simulink model "arte"  (R2013b)
settings: Solver=ode45  StartTime=0.0  StopTime=10.0  RelTol=1e-3
undefined symbols (not defined in the file or in its folder): sfp
libraries: xbsIndex_r4 x3084, casper_library_delays x44, casper_library_misc x20, dspsigops x16, xps_library x7, simulink x3
(part 1 of 27)
settings Model: Creator=root  LastModifiedBy=root
settings DebuggingCC: StateNameClashWarn=warning

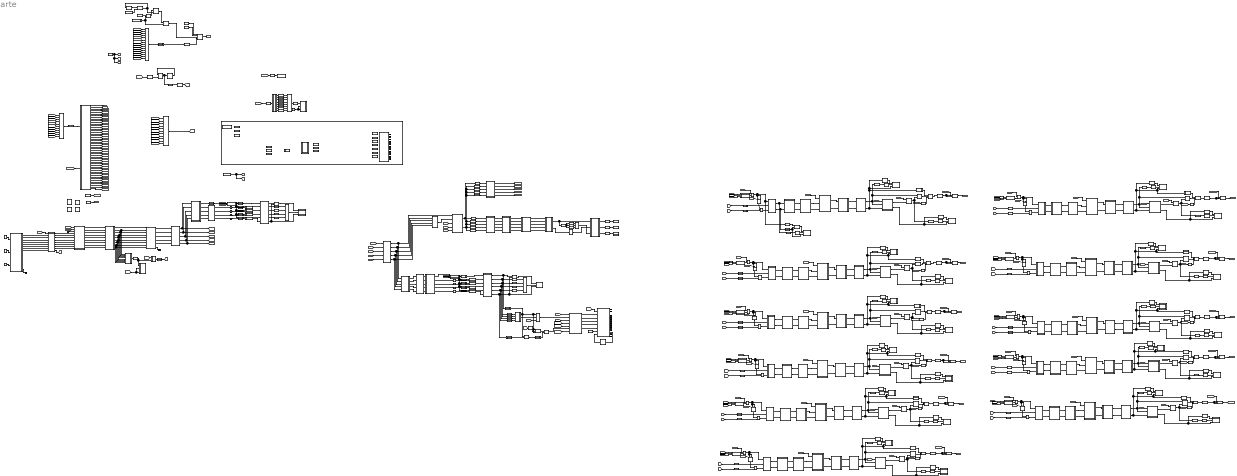
== system arte ==
  note: 5000--> 1
  note: add:3, mul:5 ->17k
  note: add:5, mul:3 ->856
  note: check if we could
      | hardcode the gain
  note: meanwhile
      | header
  note: 0xaabbccdd
  note: DRAM ring buffer + 1gbeth dump
  note: le puse un rst al contador del read!!! revisar
  " System Generator" : xbsIndex_r4/ System Generator  Tag=genX  xilinxfamily=virtex6  part=xc6vsx475t  speed=-1  package=ff1759  synthesis_tool=XST  clock_wrapper=Clock Enables  directory=./arte/sysgen  proj_type=Project Navigator  Synth_file=XST Defaults  Impl_file=ISE Defaults  testbench=off  simulink_period=1  sysclk_period=6.6667  dcm_input_clock_period=100  incr_netlist=off  trim_vbits=Everywhere in SubSystem  dbl_ovrd=According to Block Masks  core_generation=According to Block Masks  run_coregen=off  deprecated_control=off  eval_field=0  block_type=sysgen
  AddSub : xbsIndex_r4/AddSub  mode=Addition  use_carryin=off  use_carryout=off  en=off  latency=0  precision=User Defined  arith_type=Unsigned  n_bits=32  bin_pt=0  quantization=Truncate  overflow=Wrap  dbl_ovrd=off  use_behavioral_HDL=off  hw_selection=Fabric  pipelined=off  block_type=addsub
  Band-Limited White Noise : simulink/Sources/Band-Limited White Noise  Cov=[0.1]  Ts=0.1  seed=[23341]
  Band-Limited White Noise2 : simulink/Sources/Band-Limited White Noise  Cov=[0.1]  Ts=0.1  seed=[23341]
  Black Box5 : xbsIndex_r4/Black Box  init_code=fft_channel_flag_top_config  sim_method=Inactive  verbose=off  block_type=blackbox2
  Black Box6 : xbsIndex_r4/Black Box  init_code=pfb_fft_8in_2048ch_config  sim_method=Inactive  verbose=off  block_type=blackbox2
  Concat : xbsIndex_r4/Concat  num_inputs=4  dbl_ovrd=off  block_type=concat
  Concat10 : xbsIndex_r4/Concat  num_inputs=15  dbl_ovrd=off  block_type=concat
  Concat4 : xbsIndex_r4/Concat  num_inputs=4  dbl_ovrd=off  block_type=concat
  Concat5 : xbsIndex_r4/Concat  num_inputs=4  dbl_ovrd=off  block_type=concat
  Concat6 : xbsIndex_r4/Concat  num_inputs=3  dbl_ovrd=off  block_type=concat
  Concat9 : xbsIndex_r4/Concat  num_inputs=11  dbl_ovrd=off  block_type=concat
  Constant : xbsIndex_r4/Constant  const=2864434397  gui_display_data_type=Fixed-point  arith_type=Unsigned  n_bits=32  bin_pt=0  preci_type=Single  exp_width=8  frac_width=24  explicit_period=on  period=1  equ=P=C  opselect=C  inp2=PCIN>>17  opr=+  inp1=P  carry=CIN  dbl_ovrd=off  block_type=constant
  Constant1 : xbsIndex_r4/Constant  const=2864434397  gui_display_data_type=Fixed-point  arith_type=Unsigned  n_bits=32  bin_pt=0  preci_type=Single  exp_width=8  frac_width=24  explicit_period=on  period=1  equ=P=C  opselect=C  inp2=PCIN>>17  opr=+  inp1=P  carry=CIN  dbl_ovrd=off  block_type=constant
  Constant105 : xbsIndex_r4/Constant  const=1  gui_display_data_type=Boolean  arith_type=Boolean  n_bits=16  bin_pt=14  preci_type=Single  exp_width=8  frac_width=24  explicit_period=on  period=1  equ=P=C  opselect=C  inp2=PCIN>>17  opr=+  inp1=P  carry=CIN  dbl_ovrd=off  block_type=constant
  Constant13 : Constant
  Constant2 : xbsIndex_r4/Constant  const=2864434397  gui_display_data_type=Fixed-point  arith_type=Unsigned  n_bits=32  bin_pt=0  preci_type=Single  exp_width=8  frac_width=24  explicit_period=on  period=1  equ=P=C  opselect=C  inp2=PCIN>>17  opr=+  inp1=P  carry=CIN  dbl_ovrd=off  block_type=constant
  Constant3 : xbsIndex_r4/Constant  const=0  gui_display_data_type=Boolean  arith_type=Boolean  n_bits=16  bin_pt=14  preci_type=Single  exp_width=8  frac_width=24  explicit_period=on  period=1  equ=P=C  opselect=C  inp2=PCIN>>17  opr=+  inp1=P  carry=CIN  dbl_ovrd=off  block_type=constant
  Constant4 : xbsIndex_r4/Constant  const=1  gui_display_data_type=Boolean  arith_type=Boolean  n_bits=12  bin_pt=0  preci_type=Single  exp_width=8  frac_width=24  explicit_period=on  period=1  equ=P=C  opselect=C  inp2=PCIN>>17  opr=+  inp1=P  carry=CIN  dbl_ovrd=off  block_type=constant
  Constant5 : xbsIndex_r4/Constant  const=150*10^6  gui_display_data_type=Fixed-point  arith_type=Unsigned  n_bits=32  bin_pt=0  preci_type=Single  exp_width=8  frac_width=24  explicit_period=on  period=1  equ=P=C  opselect=C  inp2=PCIN>>17  opr=+  inp1=P  carry=CIN  dbl_ovrd=off  block_type=constant
  Constant6 : xbsIndex_r4/Constant  const=1  gui_display_data_type=Boolean  arith_type=Boolean  n_bits=16  bin_pt=14  preci_type=Single  exp_width=8  frac_width=24  explicit_period=on  period=1  equ=P=C  opselect=C  inp2=PCIN>>17  opr=+  inp1=P  carry=CIN  dbl_ovrd=off  block_type=constant
  Constant7 : xbsIndex_r4/Constant  const=0  gui_display_data_type=Fixed-point  arith_type=Unsigned  n_bits=32  bin_pt=0  preci_type=Single  exp_width=8  frac_width=24  explicit_period=on  period=1  equ=P=C  opselect=C  inp2=PCIN>>17  opr=+  inp1=P  carry=CIN  dbl_ovrd=off  block_type=constant
  Constant8 : xbsIndex_r4/Constant  const=1  gui_display_data_type=Boolean  arith_type=Boolean  n_bits=16  bin_pt=14  preci_type=Single  exp_width=8  frac_width=24  explicit_period=on  period=1  equ=P=C  opselect=C  inp2=PCIN>>17  opr=+  inp1=P  carry=CIN  dbl_ovrd=off  block_type=constant
  Constant9 : xbsIndex_r4/Constant  const=0  gui_display_data_type=Boolean  arith_type=Boolean  n_bits=16  bin_pt=14  preci_type=Single  exp_width=8  frac_width=24  explicit_period=on  period=1  equ=P=C  opselect=C  inp2=PCIN>>17  opr=+  inp1=P  carry=CIN  dbl_ovrd=off  block_type=constant
  Convert{1,3..4,6..13,22,31..40} (22 alike) : xbsIndex_r4/Convert  gui_display_data_type=Fixed-point  arith_type=Unsigned  n_bits=32  bin_pt=15  float_type=Single  exp_bits=8  fraction_bits=24  quantization=Truncate  overflow=Wrap  en=off  latency=0  dbl_ovrd=off  pipeline=off  block_type=convert
      settings: block_version=11.4
  Convert2 : xbsIndex_r4/Convert  gui_display_data_type=Fixed-point  arith_type="Signed  (2's comp)"  n_bits=32  bin_pt=15  float_type=Single  exp_bits=8  fraction_bits=24  quantization=Truncate  overflow=Wrap  en=off  latency=2  dbl_ovrd=off  pipeline=off  block_type=convert
      settings: block_version=11.4
  Convert{23..30} (8 alike) : xbsIndex_r4/Convert  gui_display_data_type=Fixed-point  arith_type="Signed  (2's comp)"  n_bits=8  bin_pt=0  float_type=Single  exp_bits=8  fraction_bits=24  quantization=Truncate  overflow=Wrap  en=off  latency=2  dbl_ovrd=off  pipeline=off  block_type=convert
      settings: block_version=11.4
  Convert41 : xbsIndex_r4/Convert  gui_display_data_type=Fixed-point  arith_type=Unsigned  n_bits=32  bin_pt=0  float_type=Single  exp_bits=8  fraction_bits=24  quantization=Truncate  overflow=Wrap  en=off  latency=2  dbl_ovrd=off  pipeline=off  block_type=convert
      settings: block_version=11.4
  Convert46 : xbsIndex_r4/Convert  gui_display_data_type=Boolean  arith_type=Boolean  n_bits=3  bin_pt=0  float_type=Single  exp_bits=8  fraction_bits=24  quantization=Truncate  overflow=Wrap  en=off  latency=0  dbl_ovrd=off  pipeline=off  block_type=convert
      settings: block_version=11.4
  Convert5 : xbsIndex_r4/Convert  gui_display_data_type=Boolean  arith_type=Boolean  n_bits=3  bin_pt=0  float_type=Single  exp_bits=8  fraction_bits=24  quantization=Truncate  overflow=Wrap  en=off  latency=0  dbl_ovrd=off  pipeline=off  block_type=convert
      settings: block_version=11.4
  Counter : xbsIndex_r4/Counter  cnt_type=Free Running  cnt_to=Inf  operation=Up  start_count=0  cnt_by_val=1  arith_type=Unsigned  n_bits=32  bin_pt=0  load_pin=off  rst=on  en=off  explicit_period=on  period=1  dbl_ovrd=off  use_behavioral_HDL=off  implementation=Fabric  block_type=counter
  Counter1 : xbsIndex_r4/Counter  cnt_type=Free Running  cnt_to=Inf  operation=Up  start_count=0  cnt_by_val=1  arith_type=Unsigned  n_bits=9  bin_pt=0  load_pin=off  rst=on  en=on  explicit_period=on  period=1  dbl_ovrd=off  use_behavioral_HDL=off  implementation=Fabric  block_type=counter
  Counter{8..9,12..19,21..32} (22 alike) : xbsIndex_r4/Counter  cnt_type=Free Running  cnt_to=Inf  operation=Up  start_count=0  cnt_by_val=1  arith_type=Unsigned  n_bits=10  bin_pt=0  load_pin=off  rst=off  en=on  explicit_period=on  period=1  dbl_ovrd=off  use_behavioral_HDL=off  implementation=Fabric  block_type=counter
  Counter33 : xbsIndex_r4/Counter  cnt_type=Free Running  cnt_to=Inf  operation=Up  start_count=0  cnt_by_val=1  arith_type=Unsigned  n_bits=28  bin_pt=0  load_pin=off  rst=on  en=off  explicit_period=on  period=1  dbl_ovrd=off  use_behavioral_HDL=off  implementation=Fabric  block_type=counter
  Counter34 : xbsIndex_r4/Counter  cnt_type=Free Running  cnt_to=Inf  operation=Up  start_count=0  cnt_by_val=1  arith_type=Unsigned  n_bits=32  bin_pt=0  load_pin=off  rst=on  en=on  explicit_period=on  period=1  dbl_ovrd=off  use_behavioral_HDL=off  implementation=Fabric  block_type=counter
  Counter5 : xbsIndex_r4/Counter  cnt_type=Free Running  cnt_to=Inf  operation=Up  start_count=0  cnt_by_val=1  arith_type=Unsigned  n_bits=9  bin_pt=0  load_pin=off  rst=on  en=on  explicit_period=on  period=1  dbl_ovrd=off  use_behavioral_HDL=off  implementation=Fabric  block_type=counter
  Counter6 : xbsIndex_r4/Counter  cnt_type=Free Running  cnt_to=Inf  operation=Up  start_count=0  cnt_by_val=1  arith_type=Unsigned  n_bits=3  bin_pt=0  load_pin=off  rst=on  en=off  explicit_period=on  period=1  dbl_ovrd=off  use_behavioral_HDL=off  implementation=Fabric  block_type=counter
  Counter7 : xbsIndex_r4/Counter  cnt_type=Free Running  cnt_to=Inf  operation=Up  start_count=0  cnt_by_val=1  arith_type=Unsigned  n_bits=6  bin_pt=0  load_pin=off  rst=on  en=on  explicit_period=on  period=1  dbl_ovrd=off  use_behavioral_HDL=off  implementation=Fabric  block_type=counter
  Delay{,2..5,32,34..36} (9 alike) : xbsIndex_r4/Delay  rst=off  infoeditControl=Selection of Reset will increase slice count due to use of real FFs and instead of SRLs  en=off  latency=1  dbl_ovrd=off  reg_retiming=off  block_type=delay
  Delay11 : xbsIndex_r4/Delay  rst=off  infoeditControl=Selection of Reset will increase slice count due to use of real FFs and instead of SRLs  en=off  latency=2  dbl_ovrd=off  reg_retiming=off  block_type=delay
  Delay49 : xbsIndex_r4/Delay  rst=off  infoeditControl=Selection of Reset will increase slice count due to use of real FFs and instead of SRLs  en=off  latency=2  dbl_ovrd=off  reg_retiming=off  block_type=delay
  Delay6 : xbsIndex_r4/Delay  rst=off  infoeditControl=Selection of Reset will increase slice count due to use of real FFs and instead of SRLs  en=off  latency=2  dbl_ovrd=off  reg_retiming=off  block_type=delay
  Delay91 : xbsIndex_r4/Delay  rst=off  infoeditControl=Selection of Reset will increase slice count due to use of real FFs and instead of SRLs  en=off  latency=3  dbl_ovrd=off  reg_retiming=off  block_type=delay
  Delay92 : xbsIndex_r4/Delay  rst=off  infoeditControl=Selection of Reset will increase slice count due to use of real FFs and instead of SRLs  en=off  latency=3  dbl_ovrd=off  reg_retiming=off  block_type=delay
  Delay93 : xbsIndex_r4/Delay  rst=off  infoeditControl=Selection of Reset will increase slice count due to use of real FFs and instead of SRLs  en=off  latency=3  dbl_ovrd=off  reg_retiming=off  block_type=delay
  Inverter : xbsIndex_r4/Inverter  en=off  latency=0  dbl_ovrd=off  block_type=inv
  Inverter{2,4..13} (11 alike) : xbsIndex_r4/Inverter  en=off  latency=1  dbl_ovrd=off  block_type=inv
  Inverter3 : xbsIndex_r4/Inverter  en=off  latency=0  dbl_ovrd=off  block_type=inv
  Logical : xbsIndex_r4/Logical  logical_function=OR  inputs=2  en=off  latency=0  precision=Full  arith_type=Unsigned  n_bits=16  bin_pt=0  align_bp=on  dbl_ovrd=off  block_type=logical
  Logical{1,16..22,24..27,29..30,32..33,35..36,38..39,41..42,44..45} (24 alike) : xbsIndex_r4/Logical  logical_function=AND  inputs=2  en=off  latency=0  precision=Full  arith_type=Unsigned  n_bits=16  bin_pt=0  align_bp=on  dbl_ovrd=off  block_type=logical
  Logical{2,11..15,28,31,34,37,40,43} (12 alike) : xbsIndex_r4/Logical  logical_function=AND  inputs=3  en=off  latency=0  precision=Full  arith_type=Unsigned  n_bits=16  bin_pt=0  align_bp=on  dbl_ovrd=off  block_type=logical
  Logical23 : xbsIndex_r4/Logical  logical_function=NOR  inputs=2  en=off  latency=0  precision=Full  arith_type=Unsigned  n_bits=16  bin_pt=0  align_bp=on  dbl_ovrd=off  block_type=logical
  Logical3 : xbsIndex_r4/Logical  logical_function=OR  inputs=11  en=off  latency=0  precision=Full  arith_type=Unsigned  n_bits=16  bin_pt=0  align_bp=on  dbl_ovrd=off  block_type=logical
  Model Info2 : simulink/Model-Wide Utilities/Model Info  InitialBlockCM=None  Frame=on  DisplayStringWithTags=DRAM ring buffer and 1Gbe to read  HorizontalTextAlignment=Left  LeftAlignmentValue=0.02  SourceBlockDiagram=arte  TagMaxNumber=20
  Mux : xbsIndex_r4/Mux  inputs=2  en=off  latency=1  precision=Full  arith_type=Unsigned  n_bits=16  bin_pt=14  quantization=Truncate  overflow=Wrap  dbl_ovrd=off  block_type=mux
  Register{,2..6,12..28} (23 alike) : xbsIndex_r4/Register  init=0  rst=on  en=on  dbl_ovrd=off  block_type=register
  Reinterpret : xbsIndex_r4/Reinterpret  force_arith_type=on  arith_type=Unsigned  force_bin_pt=off  bin_pt=0  block_type=reinterpret
  Reinterpret{13..16,18..20,24..26,31,33..44,49..55} (30 alike) : xbsIndex_r4/Reinterpret  force_arith_type=on  arith_type=Unsigned  force_bin_pt=on  bin_pt=0  block_type=reinterpret
  Reinterpret17 : xbsIndex_r4/Reinterpret  force_arith_type=off  arith_type=Unsigned  force_bin_pt=on  bin_pt=0  block_type=reinterpret
  Relational{,1..4,10,12..15} (10 alike) : xbsIndex_r4/Relational  mode=a>b  en=off  latency=2  dbl_ovrd=off  block_type=relational
  Relational11 : xbsIndex_r4/Relational  mode=a>b  en=off  latency=02  dbl_ovrd=off  block_type=relational
  Relational16 : xbsIndex_r4/Relational  mode=a=b  en=off  latency=0  dbl_ovrd=off  block_type=relational
  Relational17 : xbsIndex_r4/Relational  mode=a=b  en=off  latency=0  dbl_ovrd=off  block_type=relational
  Relational18 : xbsIndex_r4/Relational  mode=a=b  en=off  latency=0  dbl_ovrd=off  block_type=relational
  Shift : xbsIndex_r4/Shift  shift_dir=Left  shift_bits=11  en=off  latency=0  precision=Full  arith_type="Signed  (2's comp)"  n_bits=16  bin_pt=14  quantization=Truncate  overflow=Wrap  dbl_ovrd=off  block_type=shift
  Slice1 : xbsIndex_r4/Slice  nbits=36  boolean_output=off  mode=Lower Bit Location + Width  bit1=0  base1=MSB of Input  bit0=72  base0=LSB of Input  dbl_ovrd=off  block_type=slice
  Slice10 : xbsIndex_r4/Slice  nbits=3  boolean_output=on  mode=Lower Bit Location + Width  bit1=0  base1=MSB of Input  bit0=0  base0=LSB of Input  dbl_ovrd=off  block_type=slice
  Slice11 : xbsIndex_r4/Slice  nbits=3  boolean_output=on  mode=Lower Bit Location + Width  bit1=0  base1=MSB of Input  bit0=1  base0=LSB of Input  dbl_ovrd=off  block_type=slice
  Slice12 : xbsIndex_r4/Slice  nbits=3  boolean_output=on  mode=Lower Bit Location + Width  bit1=0  base1=MSB of Input  bit0=2  base0=LSB of Input  dbl_ovrd=off  block_type=slice
  Slice16 : xbsIndex_r4/Slice  nbits=36  boolean_output=off  mode=Lower Bit Location + Width  bit1=0  base1=MSB of Input  bit0=72  base0=LSB of Input  dbl_ovrd=off  block_type=slice
  Slice17 : xbsIndex_r4/Slice  nbits=36  boolean_output=off  mode=Lower Bit Location + Width  bit1=0  base1=MSB of Input  bit0=108  base0=LSB of Input  dbl_ovrd=off  block_type=slice
  Slice2 : xbsIndex_r4/Slice  nbits=36  boolean_output=off  mode=Lower Bit Location + Width  bit1=0  base1=MSB of Input  bit0=108  base0=LSB of Input  dbl_ovrd=off  block_type=slice
  Slice3 : xbsIndex_r4/Slice  nbits=36  boolean_output=off  mode=Lower Bit Location + Width  bit1=0  base1=MSB of Input  bit0=0  base0=LSB of Input  dbl_ovrd=off  block_type=slice
  Slice4 : xbsIndex_r4/Slice  nbits=36  boolean_output=off  mode=Lower Bit Location + Width  bit1=0  base1=MSB of Input  bit0=0  base0=LSB of Input  dbl_ovrd=off  block_type=slice
  Slice5 : xbsIndex_r4/Slice  nbits=36  boolean_output=off  mode=Lower Bit Location + Width  bit1=0  base1=MSB of Input  bit0=36  base0=LSB of Input  dbl_ovrd=off  block_type=slice
  Slice6 : xbsIndex_r4/Slice  nbits=3  boolean_output=on  mode=Lower Bit Location + Width  bit1=0  base1=MSB of Input  bit0=1  base0=LSB of Input  dbl_ovrd=off  block_type=slice
  Slice7 : xbsIndex_r4/Slice  nbits=3  boolean_output=on  mode=Lower Bit Location + Width  bit1=0  base1=MSB of Input  bit0=0  base0=LSB of Input  dbl_ovrd=off  block_type=slice
  Slice8 : xbsIndex_r4/Slice  nbits=3  boolean_output=on  mode=Lower Bit Location + Width  bit1=0  base1=MSB of Input  bit0=2  base0=LSB of Input  dbl_ovrd=off  block_type=slice
  Slice9 : xbsIndex_r4/Slice  nbits=36  boolean_output=off  mode=Lower Bit Location + Width  bit1=0  base1=MSB of Input  bit0=36  base0=LSB of Input  dbl_ovrd=off  block_type=slice
  Subsystem3 : Subsystem
  Terminator{,1,3,14..15,19..27,51..61} (25 alike) : Terminator
  XSG_core_config : xps_library/XSG_core_config  Tag=xps:xsg  hw_sys=ROACH2:sx475t  clk_src=adc0_clk  ROACH_clk_src=sys_clk  ROACH2_clk_src=adc0_clk  MKDIG_clk_src=sys_clk  clk_rate=150  sample_period=1  synthesis_tool=XST
  acc_cntrl0 : Subsystem  mask{chan_bits=9}
      mask prompts: chan_bits "Number of Channels (2^?)"
  acc_cntrl10 : Subsystem  mask{chan_bits=9}
      mask prompts: chan_bits "Number of Channels (2^?)"
  acc_cntrl11 : Subsystem  mask{chan_bits=9}
      mask prompts: chan_bits "Number of Channels (2^?)"
  acc_cntrl12 : Subsystem  mask{chan_bits=9}
      mask prompts: chan_bits "Number of Channels (2^?)"
  acc_cntrl13 : Subsystem  mask{chan_bits=9}
      mask prompts: chan_bits "Number of Channels (2^?)"
  acc_cntrl14 : Subsystem  mask{chan_bits=9}
      mask prompts: chan_bits "Number of Channels (2^?)"
  acc_cntrl15 : Subsystem  mask{chan_bits=9}
      mask prompts: chan_bits "Number of Channels (2^?)"
  acc_cntrl4 : Subsystem  mask{chan_bits=9}
      mask prompts: chan_bits "Number of Channels (2^?)"
  acc_cntrl5 : Subsystem  mask{chan_bits=9}
      mask prompts: chan_bits "Number of Channels (2^?)"
  acc_cntrl6 : Subsystem  mask{chan_bits=9}
      mask prompts: chan_bits "Number of Channels (2^?)"
  acc_cntrl7 : Subsystem  mask{chan_bits=9}
      mask prompts: chan_bits "Number of Channels (2^?)"
  acc_cntrl8 : Subsystem  mask{chan_bits=9}
      mask prompts: chan_bits "Number of Channels (2^?)"
  acc_cntrl9 : Subsystem  mask{chan_bits=9}
      mask prompts: chan_bits "Number of Channels (2^?)"
  adc_clip0 : Subsystem
  adcsnap0 : Subsystem  Tag=casper:snapshot  AncestorBlock=casper_library_scopes/snapshot  mask(snapshot){storage=bram, dram_dimm=1, dram_clock=200, nsamples=10, data_width=64, offset=on, circap=off, value=off, use_dsp48=off}
      mask prompts: storage "Storage medium"; dram_dimm "DRAM dimm"; dram_clock "DRAM clock rate"; nsamples "Number of Samples (2^?)"; data_width "Data width"; offset "Start delay support"; circap "Circular capture support"; value "Extra value capture support"; use_dsp48 "Use DSP48s to implement counters"
      mask help:
      | Standard snap block, but with the following optional extras;
      |  1) Optionally delay the fabric trigger by a user-specified number of valids.
      |  2) Capture continuously after a trigger until a stop pulse is received. Data is captured into BRAM continuously, with old data being overwritten until a stop command is received. Then stop capturing when memory is filled. This enables you to get some data before and some data after the stop pulse. Use the 'tr_en_cnt' register to determine where you are in your vector. 'Addr' register's MSb now indicates 'busy capturing'.
      |  3) Optionally capture a value on an input port to a register at the same time as the first data sample.
      |  4) Implement counters using DSP48Es to save resources.
      mask init:
      | snapshot_init(gcb, ...
      |     'storage', storage, ...
      |     'dram_dimm', dram_dimm, ...
      |     'dram_clock', dram_clock, ...
      |     'nsamples', nsamples, ...
      |     'data_width', data_width, ...
      |     'offset', offset, ...
      |     'circap', circap, ...
      |     'value', value, ...
      |     'use_dsp48', use_dsp48);
      mask TypeOptions storage: bram | dram
      mask Callback storage: snapshot_callback();
      mask TypeOptions dram_dimm: 1 | 2 | 3 | 4
      mask TypeOptions dram_clock: 200 | 250 | 266 | 300 | 333
      mask TypeOptions data_width: 8 | 16 | 32 | 64 | 128
  add_stat{0..10} (11 alike) : xbsIndex_r4/AddSub  mode=Addition  use_carryin=off  use_carryout=off  en=off  latency=1  precision=User Defined  arith_type=Unsigned  n_bits=25  bin_pt=15  quantization=Truncate  overflow=Wrap  dbl_ovrd=off  use_behavioral_HDL=off  hw_selection=Fabric  pipelined=off  block_type=addsub
  adder_tree1 : Subsystem  AncestorBlock=casper_library_misc/adder_tree  mask(adder_tree){n_inputs=4, latency=1, adder_imp=Fabric, first_stage_hdl=on}
      mask prompts: n_inputs "Number of Inputs"; latency "Add Latency"; adder_imp "Adder implementation"; first_stage_hdl "Use behavioural HDL for first stage of adders"
      mask help:
      | Sums all inputs using a tree of adds and delays.
      |
      | Number of inputs: The number of inputs to the block to be summed
      | Add latency: The number of clock cycles to perform one addition (affects timing)..
      | Adder implementation: choice of fabric or DSP48E core, or behavioral HDL
      | Use behavioural HDL for first stage of adders: Causes the first stage of adders to be absorbed into DSP blocks if multipliers precede them (Virtex 5). Overrides Adder implementation
      mask init:
      | adder_tree_init(gcb, ...
      |     'n_inputs', n_inputs, ...
      |     'latency', latency, ...
      |     'adder_imp', adder_imp, ...
      |     'first_stage_hdl', first_stage_hdl);
      settings: AttributesFormatString=latency 2
      mask Help: eval('xlWeb(''http://casper.berkeley.edu/wiki/Adder_tree'')')
      mask TypeOptions adder_imp: Behavioral | Fabric | DSP48
  antenna_0 : Subsystem  Tag=xps:bram  AncestorBlock=xps_library/Shared_BRAM  mask{arith_type=Unsigned, addr_width=9, data_width=128, reg_prim_output=off, reg_core_output=off, optimization=Minimum_Area, data_bin_pt=0, init_vals=[0:2^10-1], sample_rate=1}
      mask prompts: arith_type "Output Data Type"; addr_width "Address width"; data_width "Data Width"; reg_prim_output "Register Primitive Output"; reg_core_output "Register Core Output"; data_bin_pt "Data Binary Point"; init_vals "Initial values (simulation only)"; sample_rate "Sample rate"
      mask init:
      | shared_bram_mask;
      mask TypeOptions arith_type: Unsigned | Signed  (2's comp)
      mask TypeOptions data_width: 8 | 16 | 32 | 64 | 128
      mask TypeOptions optimization: Minimum_Area | Low_Power
  antenna_power0 : Subsystem  mask{add_lat=2, mult_lat=3}
  asiaa_adc5g0 : Subsystem  Tag=xps:adc5g  AncestorBlock=xps_library/ADCs/asiaa_adc5g  mask(adc5g){input_mode=Two-channel -- A&C, adc_brd=ZDOK 0, demux=1:1, adc_bit_width=8, adc_clk_rate=1200, using_ctrl=on, test_ramp=off}
      mask prompts: input_mode "Input mode:"; adc_brd "ADC Board"; demux "Internal demux"; adc_bit_width "ADC Resolution (bits):"; adc_clk_rate "ADC Clock Rate (MHz):"; using_ctrl "use control"; test_ramp "start in test ramp mode"
      mask help:
      | Interface for the ASIAA 5 GSps ADC. Supports interleaving all four
      | cores using either input A or C, or interleaving two-cores each for
      | A and C. The hardware itself comes in two versions:
      |
      | DMUX 1:2 -- 4-bit samples, 4 parallel streams
      | DMUX 1:1 -- 8-bit samples, 2 parallel streams
      |
      | In either configuration this block will output 8 parallel streams
      | but the underlying interface, and the bitwidth of the samples,
      | will be different.
      mask init:
      | adc5g_init(gcb,...
      |     'input_mode', input_mode,...
      |     'demux', demux,...
      |     'adc_clk_rate', adc_clk_rate,...
      |     'adc_bit_width', adc_bit_width,...
      |     'adc_brd', adc_brd,...
      |     'using_ctrl', using_ctrl,...
      |     'test_ramp', test_ramp);
      mask TypeOptions input_mode: One-channel -- A | One-channel -- C | Two-channel -- A&C
      mask TypeOptions adc_brd: ZDOK 0 | ZDOK 1
      mask TypeOptions demux: 1:1 | 1:2
      mask Callback demux:
      | demux = get_param(gcb,'demux');
      | if(strcmp(demux,'1:1')),
      |     set_param(gcb, 'adc_bit_width', '8')
      | elseif(strcmp(demux, '1:2')),
      |     set_param(gcb, 'adc_bit_width', '4');
      | else
      | end
  avg0 : Subsystem  Tag=xps:bram  AncestorBlock=xps_library/Shared_BRAM  mask{arith_type=Unsigned, addr_width=10, data_width=32, reg_prim_output=off, reg_core_output=off, optimization=Minimum_Area, data_bin_pt=0, init_vals=[0:2^10-1], sample_rate=1}
      mask prompts: arith_type "Output Data Type"; addr_width "Address width"; data_width "Data Width"; reg_prim_output "Register Primitive Output"; reg_core_output "Register Core Output"; data_bin_pt "Data Binary Point"; init_vals "Initial values (simulation only)"; sample_rate "Sample rate"
      mask init:
      | shared_bram_mask;
      mask TypeOptions arith_type: Unsigned | Signed  (2's comp)
      mask TypeOptions data_width: 8 | 16 | 32 | 64 | 128
      mask TypeOptions optimization: Minimum_Area | Low_Power
  avg1 : Subsystem  Tag=xps:bram  AncestorBlock=xps_library/Shared_BRAM  mask{arith_type=Unsigned, addr_width=10, data_width=32, reg_prim_output=off, reg_core_output=off, optimization=Minimum_Area, data_bin_pt=0, init_vals=[0:2^10-1], sample_rate=1}
      mask prompts: arith_type "Output Data Type"; addr_width "Address width"; data_width "Data Width"; reg_prim_output "Register Primitive Output"; reg_core_output "Register Core Output"; data_bin_pt "Data Binary Point"; init_vals "Initial values (simulation only)"; sample_rate "Sample rate"
      mask init:
      | shared_bram_mask;
      mask TypeOptions arith_type: Unsigned | Signed  (2's comp)
      mask TypeOptions data_width: 8 | 16 | 32 | 64 | 128
      mask TypeOptions optimization: Minimum_Area | Low_Power
  avg10 : Subsystem  Tag=xps:bram  AncestorBlock=xps_library/Shared_BRAM  mask{arith_type=Unsigned, addr_width=10, data_width=32, reg_prim_output=off, reg_core_output=off, optimization=Minimum_Area, data_bin_pt=0, init_vals=[0:2^10-1], sample_rate=1}
      mask prompts: arith_type "Output Data Type"; addr_width "Address width"; data_width "Data Width"; reg_prim_output "Register Primitive Output"; reg_core_output "Register Core Output"; data_bin_pt "Data Binary Point"; init_vals "Initial values (simulation only)"; sample_rate "Sample rate"
      mask init:
      | shared_bram_mask;
      mask TypeOptions arith_type: Unsigned | Signed  (2's comp)
      mask TypeOptions data_width: 8 | 16 | 32 | 64 | 128
      mask TypeOptions optimization: Minimum_Area | Low_Power
  avg2 : Subsystem  Tag=xps:bram  AncestorBlock=xps_library/Shared_BRAM  mask{arith_type=Unsigned, addr_width=10, data_width=32, reg_prim_output=off, reg_core_output=off, optimization=Minimum_Area, data_bin_pt=0, init_vals=[0:2^10-1], sample_rate=1}
      mask prompts: arith_type "Output Data Type"; addr_width "Address width"; data_width "Data Width"; reg_prim_output "Register Primitive Output"; reg_core_output "Register Core Output"; data_bin_pt "Data Binary Point"; init_vals "Initial values (simulation only)"; sample_rate "Sample rate"
      mask init:
      | shared_bram_mask;
      mask TypeOptions arith_type: Unsigned | Signed  (2's comp)
      mask TypeOptions data_width: 8 | 16 | 32 | 64 | 128
      mask TypeOptions optimization: Minimum_Area | Low_Power
  avg3 : Subsystem  Tag=xps:bram  AncestorBlock=xps_library/Shared_BRAM  mask{arith_type=Unsigned, addr_width=10, data_width=32, reg_prim_output=off, reg_core_output=off, optimization=Minimum_Area, data_bin_pt=0, init_vals=[0:2^10-1], sample_rate=1}
      mask prompts: arith_type "Output Data Type"; addr_width "Address width"; data_width "Data Width"; reg_prim_output "Register Primitive Output"; reg_core_output "Register Core Output"; data_bin_pt "Data Binary Point"; init_vals "Initial values (simulation only)"; sample_rate "Sample rate"
      mask init:
      | shared_bram_mask;
      mask TypeOptions arith_type: Unsigned | Signed  (2's comp)
      mask TypeOptions data_width: 8 | 16 | 32 | 64 | 128
      mask TypeOptions optimization: Minimum_Area | Low_Power
  avg4 : Subsystem  Tag=xps:bram  AncestorBlock=xps_library/Shared_BRAM  mask{arith_type=Unsigned, addr_width=10, data_width=32, reg_prim_output=off, reg_core_output=off, optimization=Minimum_Area, data_bin_pt=0, init_vals=[0:2^10-1], sample_rate=1}
      mask prompts: arith_type "Output Data Type"; addr_width "Address width"; data_width "Data Width"; reg_prim_output "Register Primitive Output"; reg_core_output "Register Core Output"; data_bin_pt "Data Binary Point"; init_vals "Initial values (simulation only)"; sample_rate "Sample rate"
      mask init:
      | shared_bram_mask;
      mask TypeOptions arith_type: Unsigned | Signed  (2's comp)
      mask TypeOptions data_width: 8 | 16 | 32 | 64 | 128
      mask TypeOptions optimization: Minimum_Area | Low_Power
  avg5 : Subsystem  Tag=xps:bram  AncestorBlock=xps_library/Shared_BRAM  mask{arith_type=Unsigned, addr_width=10, data_width=32, reg_prim_output=off, reg_core_output=off, optimization=Minimum_Area, data_bin_pt=0, init_vals=[0:2^10-1], sample_rate=1}
      mask prompts: arith_type "Output Data Type"; addr_width "Address width"; data_width "Data Width"; reg_prim_output "Register Primitive Output"; reg_core_output "Register Core Output"; data_bin_pt "Data Binary Point"; init_vals "Initial values (simulation only)"; sample_rate "Sample rate"
      mask init:
      | shared_bram_mask;
      mask TypeOptions arith_type: Unsigned | Signed  (2's comp)
      mask TypeOptions data_width: 8 | 16 | 32 | 64 | 128
      mask TypeOptions optimization: Minimum_Area | Low_Power
  avg6 : Subsystem  Tag=xps:bram  AncestorBlock=xps_library/Shared_BRAM  mask{arith_type=Unsigned, addr_width=10, data_width=32, reg_prim_output=off, reg_core_output=off, optimization=Minimum_Area, data_bin_pt=0, init_vals=[0:2^10-1], sample_rate=1}
      mask prompts: arith_type "Output Data Type"; addr_width "Address width"; data_width "Data Width"; reg_prim_output "Register Primitive Output"; reg_core_output "Register Core Output"; data_bin_pt "Data Binary Point"; init_vals "Initial values (simulation only)"; sample_rate "Sample rate"
      mask init:
      | shared_bram_mask;
      mask TypeOptions arith_type: Unsigned | Signed  (2's comp)
      mask TypeOptions data_width: 8 | 16 | 32 | 64 | 128
      mask TypeOptions optimization: Minimum_Area | Low_Power
  avg7 : Subsystem  Tag=xps:bram  AncestorBlock=xps_library/Shared_BRAM  mask{arith_type=Unsigned, addr_width=10, data_width=32, reg_prim_output=off, reg_core_output=off, optimization=Minimum_Area, data_bin_pt=0, init_vals=[0:2^10-1], sample_rate=1}
      mask prompts: arith_type "Output Data Type"; addr_width "Address width"; data_width "Data Width"; reg_prim_output "Register Primitive Output"; reg_core_output "Register Core Output"; data_bin_pt "Data Binary Point"; init_vals "Initial values (simulation only)"; sample_rate "Sample rate"
      mask init:
      | shared_bram_mask;
      mask TypeOptions arith_type: Unsigned | Signed  (2's comp)
      mask TypeOptions data_width: 8 | 16 | 32 | 64 | 128
      mask TypeOptions optimization: Minimum_Area | Low_Power
  avg8 : Subsystem  Tag=xps:bram  AncestorBlock=xps_library/Shared_BRAM  mask{arith_type=Unsigned, addr_width=10, data_width=32, reg_prim_output=off, reg_core_output=off, optimization=Minimum_Area, data_bin_pt=0, init_vals=[0:2^10-1], sample_rate=1}
      mask prompts: arith_type "Output Data Type"; addr_width "Address width"; data_width "Data Width"; reg_prim_output "Register Primitive Output"; reg_core_output "Register Core Output"; data_bin_pt "Data Binary Point"; init_vals "Initial values (simulation only)"; sample_rate "Sample rate"
      mask init:
      | shared_bram_mask;
      mask TypeOptions arith_type: Unsigned | Signed  (2's comp)
      mask TypeOptions data_width: 8 | 16 | 32 | 64 | 128
      mask TypeOptions optimization: Minimum_Area | Low_Power
  avg9 : Subsystem  Tag=xps:bram  AncestorBlock=xps_library/Shared_BRAM  mask{arith_type=Unsigned, addr_width=10, data_width=32, reg_prim_output=off, reg_core_output=off, optimization=Minimum_Area, data_bin_pt=0, init_vals=[0:2^10-1], sample_rate=1}
      mask prompts: arith_type "Output Data Type"; addr_width "Address width"; data_width "Data Width"; reg_prim_output "Register Primitive Output"; reg_core_output "Register Core Output"; data_bin_pt "Data Binary Point"; init_vals "Initial values (simulation only)"; sample_rate "Sample rate"
      mask init:
      | shared_bram_mask;
      mask TypeOptions arith_type: Unsigned | Signed  (2's comp)
      mask TypeOptions data_width: 8 | 16 | 32 | 64 | 128
      mask TypeOptions optimization: Minimum_Area | Low_Power
  beam : Subsystem  Tag=xps:bram  AncestorBlock=xps_library/Shared_BRAM  mask{arith_type=Unsigned, addr_width=9, data_width=128, reg_prim_output=off, reg_core_output=off, optimization=Minimum_Area, data_bin_pt=0, init_vals=[0:2^10-1], sample_rate=1}
      mask prompts: arith_type "Output Data Type"; addr_width "Address width"; data_width "Data Width"; reg_prim_output "Register Primitive Output"; reg_core_output "Register Core Output"; data_bin_pt "Data Binary Point"; init_vals "Initial values (simulation only)"; sample_rate "Sample rate"
      mask init:
      | shared_bram_mask;
      mask TypeOptions arith_type: Unsigned | Signed  (2's comp)
      mask TypeOptions data_width: 8 | 16 | 32 | 64 | 128
      mask TypeOptions optimization: Minimum_Area | Low_Power
  beam_post_acc_delay : Subsystem  mask{lat=2}
  beam_post_complex_add : Subsystem  mask{lat=3}
  beam_power : Subsystem  mask{add_lat=4, mult_lat=4}
  beam_power_conv : Subsystem  mask{shift_val=15, conv_width=16, conv_point=15}
      mask prompts: shift_val "shift"; conv_width "convert width"; conv_point "convert point"
  beam_rfi_delay : Subsystem  mask{lat=3}
  beam_vacc0 : Subsystem  AncestorBlock=casper_library_accumulators/simple_bram_vacc  mask(simple_bram_vacc){vec_len=512, arith_type=Unsigned, n_bits=32, bin_pt=15}
      mask prompts: vec_len "Vector length:"; arith_type "Output type:"; n_bits "Bit width (output):"; bin_pt "Binary point (output):"
      mask help: This simple vector accumulator is based on a shift register. It outputs its previous accumulated vector after a new_acc pulse is received.
      mask init:
      | simple_bram_vacc_init(gcb, ...
      |     'vec_len', vec_len, ...
      |     'arith_type', arith_type, ...
      |     'n_bits', n_bits, ...
      |     'bin_pt', bin_pt);
      mask TypeOptions arith_type: Signed | Unsigned
  beam_vacc1 : Subsystem  AncestorBlock=casper_library_accumulators/simple_bram_vacc  mask(simple_bram_vacc){vec_len=512, arith_type=Unsigned, n_bits=32, bin_pt=15}
      mask prompts: vec_len "Vector length:"; arith_type "Output type:"; n_bits "Bit width (output):"; bin_pt "Binary point (output):"
      mask help: This simple vector accumulator is based on a shift register. It outputs its previous accumulated vector after a new_acc pulse is received.
      mask init:
      | simple_bram_vacc_init(gcb, ...
      |     'vec_len', vec_len, ...
      |     'arith_type', arith_type, ...
      |     'n_bits', n_bits, ...
      |     'bin_pt', bin_pt);
      mask TypeOptions arith_type: Signed | Unsigned
  beam_vacc2 : Subsystem  AncestorBlock=casper_library_accumulators/simple_bram_vacc  mask(simple_bram_vacc){vec_len=512, arith_type=Unsigned, n_bits=32, bin_pt=15}
      mask prompts: vec_len "Vector length:"; arith_type "Output type:"; n_bits "Bit width (output):"; bin_pt "Binary point (output):"
      mask help: This simple vector accumulator is based on a shift register. It outputs its previous accumulated vector after a new_acc pulse is received.
      mask init:
      | simple_bram_vacc_init(gcb, ...
      |     'vec_len', vec_len, ...
      |     'arith_type', arith_type, ...
      |     'n_bits', n_bits, ...
      |     'bin_pt', bin_pt);
      mask TypeOptions arith_type: Signed | Unsigned
  beam_vacc3 : Subsystem  AncestorBlock=casper_library_accumulators/simple_bram_vacc  mask(simple_bram_vacc){vec_len=512, arith_type=Unsigned, n_bits=32, bin_pt=15}
      mask prompts: vec_len "Vector length:"; arith_type "Output type:"; n_bits "Bit width (output):"; bin_pt "Binary point (output):"
      mask help: This simple vector accumulator is based on a shift register. It outputs its previous accumulated vector after a new_acc pulse is received.
      mask init:
      | simple_bram_vacc_init(gcb, ...
      |     'vec_len', vec_len, ...
      |     'arith_type', arith_type, ...
      |     'n_bits', n_bits, ...
      |     'bin_pt', bin_pt);
      mask TypeOptions arith_type: Signed | Unsigned
  bus_create : Subsystem  AncestorBlock=casper_library_flow_control/bus_create  mask(bus_create){inputNum=8}
      mask prompts: inputNum "Number of inputs:"
      mask init:
      | bus_create_init(gcb,...
      |     'inputNum', inputNum);
  bus_create4 : Subsystem  AncestorBlock=casper_library_flow_control/bus_create  mask(bus_create){inputNum=8}
      mask prompts: inputNum "Number of inputs:"
      mask init:
      | bus_create_init(gcb,...
      |     'inputNum', inputNum);
  bus_expand : Subsystem  AncestorBlock=casper_library_flow_control/bus_expand  mask(bus_expand){mode=divisions of equal size, outputNum=8, outputWidth=4, outputBinaryPt=0, outputArithmeticType=1, show_format=off, outputToWorkspace=off, variablePrefix=out, outputToModelAsWell=on}
      mask prompts: outputNum "Number of outputs:"; outputWidth "Output width:"; outputBinaryPt "Output binary point position:"; outputArithmeticType "Output arithmetic type (ufix=0, fix=1, bool=2):"; show_format "Print format string?"; outputToWorkspace "Output to workspace?"; variablePrefix "Variable name prefix:"; outputToModelAsWell "Output to model as well?"
      mask help:
      | Expands a 'bus' made using a bus_create or Xilinx
      | concat block.
      | The input will be divided into the specified number
      | of outputs with the specified arithmetic types.
      | Divisions are made from most significant bit.
      mask init:
      | bus_expand_init(gcb,...
      |     'mode', mode, ...
      |     'outputNum', outputNum, ...
      |     'outputWidth', outputWidth, ...
      |     'outputBinaryPt', outputBinaryPt, ...
      |     'outputArithmeticType', outputArithmeticType, ...
      |     'show_format', show_format, ...
      |     'outputToWorkspace', outputToWorkspace, ...
      |     'variablePrefix', variablePrefix, ...
      |     'outputToModelAsWell', outputToModelAsWell);
      settings: AttributesFormatString=8 outputs
      mask TypeOptions mode: divisions of equal size | divisions of arbitrary size
      mask Callback mode: bus_expand_callback();
      mask Callback outputWidth: bus_expand_callback();
      mask Callback outputToWorkspace: bus_expand_callback();
  concat_ : Subsystem
  concat_order : Subsystem
  control : Subsystem
  control1 : Subsystem  Tag=xps:sw_reg  AncestorBlock=xps_library/software_register  mask(swreg){io_dir=From Processor, io_delay=0, sample_period=1, names=reg, bitwidths=32, bin_pts=0, arith_types=0, sim_port=off, show_format=on}
      mask prompts: io_dir "I/O direction"; io_delay "I/O delay"; sample_period "Sample period"; names "Bitfield names [msb...lsb]"; bitwidths "Bitfield widths"; bin_pts "Bitfield binary pts"; arith_types "Bitfield types, ufix=0, fix=1, bool=2"; sim_port "Provide sim input/output?"; show_format "Print format string?"
      mask help: A 32-bit software-accessible register. Can be divided into bitfields of varying widths and types using the fields in the block mask.
      mask init:
      | try
      |     swreg_init(gcb)
      | catch ex
      |     disp(sprintf('%s: %s', gcb, ex.message))
      |     errordlg(ex.message)
      | end
      settings: AttributesFormatString=1input:uf32.0 = 32 bits
      mask TypeOptions io_dir: To Processor | From Processor
      mask Callback io_dir:
      | mask_enables = get_param(gcb, 'MaskEnables');
      | mask_names = get_param(gcb, 'MaskNames');
      | if strcmp(get_param(gcb, 'io_dir'), 'To Processor'),
      |     mask_enables{ismember(mask_names, 'sample_period')} = 'off';
      | else
      |     mask_enables{ismember(mask_names, 'sample_period')} = 'on';
      | end
      | set_param(gcb, 'MaskEnables', mask_enables);
  conv_bus4 : Subsystem
  debug_acc : Subsystem  Tag=xps:bram  AncestorBlock=xps_library/Shared_BRAM  mask{arith_type=Unsigned, addr_width=10, data_width=32, reg_prim_output=off, reg_core_output=off, optimization=Minimum_Area, data_bin_pt=0, init_vals=[0:2^10-1], sample_rate=1}
      mask prompts: arith_type "Output Data Type"; addr_width "Address width"; data_width "Data Width"; reg_prim_output "Register Primitive Output"; reg_core_output "Register Core Output"; data_bin_pt "Data Binary Point"; init_vals "Initial values (simulation only)"; sample_rate "Sample rate"
      mask init:
      | shared_bram_mask;
      mask TypeOptions arith_type: Unsigned | Signed  (2's comp)
      mask TypeOptions data_width: 8 | 16 | 32 | 64 | 128
      mask TypeOptions optimization: Minimum_Area | Low_Power
  dedisp0 : Subsystem  Tag=xps:bram  AncestorBlock=xps_library/Shared_BRAM  mask{arith_type=Unsigned, addr_width=10, data_width=32, reg_prim_output=off, reg_core_output=off, optimization=Minimum_Area, data_bin_pt=0, init_vals=[0:2^10-1], sample_rate=1}
      mask prompts: arith_type "Output Data Type"; addr_width "Address width"; data_width "Data Width"; reg_prim_output "Register Primitive Output"; reg_core_output "Register Core Output"; data_bin_pt "Data Binary Point"; init_vals "Initial values (simulation only)"; sample_rate "Sample rate"
      mask init:
      | shared_bram_mask;
      mask TypeOptions arith_type: Unsigned | Signed  (2's comp)
      mask TypeOptions data_width: 8 | 16 | 32 | 64 | 128
      mask TypeOptions optimization: Minimum_Area | Low_Power
  dedisp1 : Subsystem  Tag=xps:bram  AncestorBlock=xps_library/Shared_BRAM  mask{arith_type=Unsigned, addr_width=10, data_width=32, reg_prim_output=off, reg_core_output=off, optimization=Minimum_Area, data_bin_pt=0, init_vals=[0:2^10-1], sample_rate=1}
      mask prompts: arith_type "Output Data Type"; addr_width "Address width"; data_width "Data Width"; reg_prim_output "Register Primitive Output"; reg_core_output "Register Core Output"; data_bin_pt "Data Binary Point"; init_vals "Initial values (simulation only)"; sample_rate "Sample rate"
      mask init:
      | shared_bram_mask;
      mask TypeOptions arith_type: Unsigned | Signed  (2's comp)
      mask TypeOptions data_width: 8 | 16 | 32 | 64 | 128
      mask TypeOptions optimization: Minimum_Area | Low_Power
  dedisp10 : Subsystem  Tag=xps:bram  AncestorBlock=xps_library/Shared_BRAM  mask{arith_type=Unsigned, addr_width=10, data_width=32, reg_prim_output=off, reg_core_output=off, optimization=Minimum_Area, data_bin_pt=0, init_vals=[0:2^10-1], sample_rate=1}
      mask prompts: arith_type "Output Data Type"; addr_width "Address width"; data_width "Data Width"; reg_prim_output "Register Primitive Output"; reg_core_output "Register Core Output"; data_bin_pt "Data Binary Point"; init_vals "Initial values (simulation only)"; sample_rate "Sample rate"
      mask init:
      | shared_bram_mask;
      mask TypeOptions arith_type: Unsigned | Signed  (2's comp)
      mask TypeOptions data_width: 8 | 16 | 32 | 64 | 128
      mask TypeOptions optimization: Minimum_Area | Low_Power
  dedisp2 : Subsystem  Tag=xps:bram  AncestorBlock=xps_library/Shared_BRAM  mask{arith_type=Unsigned, addr_width=10, data_width=32, reg_prim_output=off, reg_core_output=off, optimization=Minimum_Area, data_bin_pt=0, init_vals=[0:2^10-1], sample_rate=1}
      mask prompts: arith_type "Output Data Type"; addr_width "Address width"; data_width "Data Width"; reg_prim_output "Register Primitive Output"; reg_core_output "Register Core Output"; data_bin_pt "Data Binary Point"; init_vals "Initial values (simulation only)"; sample_rate "Sample rate"
      mask init:
      | shared_bram_mask;
      mask TypeOptions arith_type: Unsigned | Signed  (2's comp)
      mask TypeOptions data_width: 8 | 16 | 32 | 64 | 128
      mask TypeOptions optimization: Minimum_Area | Low_Power
  dedisp3 : Subsystem  Tag=xps:bram  AncestorBlock=xps_library/Shared_BRAM  mask{arith_type=Unsigned, addr_width=10, data_width=32, reg_prim_output=off, reg_core_output=off, optimization=Minimum_Area, data_bin_pt=0, init_vals=[0:2^10-1], sample_rate=1}
      mask prompts: arith_type "Output Data Type"; addr_width "Address width"; data_width "Data Width"; reg_prim_output "Register Primitive Output"; reg_core_output "Register Core Output"; data_bin_pt "Data Binary Point"; init_vals "Initial values (simulation only)"; sample_rate "Sample rate"
      mask init:
      | shared_bram_mask;
      mask TypeOptions arith_type: Unsigned | Signed  (2's comp)
      mask TypeOptions data_width: 8 | 16 | 32 | 64 | 128
      mask TypeOptions optimization: Minimum_Area | Low_Power
  dedisp4 : Subsystem  Tag=xps:bram  AncestorBlock=xps_library/Shared_BRAM  mask{arith_type=Unsigned, addr_width=10, data_width=32, reg_prim_output=off, reg_core_output=off, optimization=Minimum_Area, data_bin_pt=0, init_vals=[0:2^10-1], sample_rate=1}
      mask prompts: arith_type "Output Data Type"; addr_width "Address width"; data_width "Data Width"; reg_prim_output "Register Primitive Output"; reg_core_output "Register Core Output"; data_bin_pt "Data Binary Point"; init_vals "Initial values (simulation only)"; sample_rate "Sample rate"
      mask init:
      | shared_bram_mask;
      mask TypeOptions arith_type: Unsigned | Signed  (2's comp)
      mask TypeOptions data_width: 8 | 16 | 32 | 64 | 128
      mask TypeOptions optimization: Minimum_Area | Low_Power
  dedisp5 : Subsystem  Tag=xps:bram  AncestorBlock=xps_library/Shared_BRAM  mask{arith_type=Unsigned, addr_width=10, data_width=32, reg_prim_output=off, reg_core_output=off, optimization=Minimum_Area, data_bin_pt=0, init_vals=[0:2^10-1], sample_rate=1}
      mask prompts: arith_type "Output Data Type"; addr_width "Address width"; data_width "Data Width"; reg_prim_output "Register Primitive Output"; reg_core_output "Register Core Output"; data_bin_pt "Data Binary Point"; init_vals "Initial values (simulation only)"; sample_rate "Sample rate"
      mask init:
      | shared_bram_mask;
      mask TypeOptions arith_type: Unsigned | Signed  (2's comp)
      mask TypeOptions data_width: 8 | 16 | 32 | 64 | 128
      mask TypeOptions optimization: Minimum_Area | Low_Power
  dedisp6 : Subsystem  Tag=xps:bram  AncestorBlock=xps_library/Shared_BRAM  mask{arith_type=Unsigned, addr_width=10, data_width=32, reg_prim_output=off, reg_core_output=off, optimization=Minimum_Area, data_bin_pt=0, init_vals=[0:2^10-1], sample_rate=1}
      mask prompts: arith_type "Output Data Type"; addr_width "Address width"; data_width "Data Width"; reg_prim_output "Register Primitive Output"; reg_core_output "Register Core Output"; data_bin_pt "Data Binary Point"; init_vals "Initial values (simulation only)"; sample_rate "Sample rate"
      mask init:
      | shared_bram_mask;
      mask TypeOptions arith_type: Unsigned | Signed  (2's comp)
      mask TypeOptions data_width: 8 | 16 | 32 | 64 | 128
      mask TypeOptions optimization: Minimum_Area | Low_Power
  dedisp7 : Subsystem  Tag=xps:bram  AncestorBlock=xps_library/Shared_BRAM  mask{arith_type=Unsigned, addr_width=10, data_width=32, reg_prim_output=off, reg_core_output=off, optimization=Minimum_Area, data_bin_pt=0, init_vals=[0:2^10-1], sample_rate=1}
      mask prompts: arith_type "Output Data Type"; addr_width "Address width"; data_width "Data Width"; reg_prim_output "Register Primitive Output"; reg_core_output "Register Core Output"; data_bin_pt "Data Binary Point"; init_vals "Initial values (simulation only)"; sample_rate "Sample rate"
      mask init:
      | shared_bram_mask;
      mask TypeOptions arith_type: Unsigned | Signed  (2's comp)
      mask TypeOptions data_width: 8 | 16 | 32 | 64 | 128
      mask TypeOptions optimization: Minimum_Area | Low_Power
  dedisp8 : Subsystem  Tag=xps:bram  AncestorBlock=xps_library/Shared_BRAM  mask{arith_type=Unsigned, addr_width=10, data_width=32, reg_prim_output=off, reg_core_output=off, optimization=Minimum_Area, data_bin_pt=0, init_vals=[0:2^10-1], sample_rate=1}
      mask prompts: arith_type "Output Data Type"; addr_width "Address width"; data_width "Data Width"; reg_prim_output "Register Primitive Output"; reg_core_output "Register Core Output"; data_bin_pt "Data Binary Point"; init_vals "Initial values (simulation only)"; sample_rate "Sample rate"
      mask init:
      | shared_bram_mask;
      mask TypeOptions arith_type: Unsigned | Signed  (2's comp)
      mask TypeOptions data_width: 8 | 16 | 32 | 64 | 128
      mask TypeOptions optimization: Minimum_Area | Low_Power
  dedisp9 : Subsystem  Tag=xps:bram  AncestorBlock=xps_library/Shared_BRAM  mask{arith_type=Unsigned, addr_width=10, data_width=32, reg_prim_output=off, reg_core_output=off, optimization=Minimum_Area, data_bin_pt=0, init_vals=[0:2^10-1], sample_rate=1}
      mask prompts: arith_type "Output Data Type"; addr_width "Address width"; data_width "Data Width"; reg_prim_output "Register Primitive Output"; reg_core_output "Register Core Output"; data_bin_pt "Data Binary Point"; init_vals "Initial values (simulation only)"; sample_rate "Sample rate"
      mask init:
      | shared_bram_mask;
      mask TypeOptions arith_type: Unsigned | Signed  (2's comp)
      mask TypeOptions data_width: 8 | 16 | 32 | 64 | 128
      mask TypeOptions optimization: Minimum_Area | Low_Power
  dedispersor0 : Subsystem  mask{din_width=25, din_point=15, dout_width=25}
      mask prompts: din_width "Input width"; din_point "Input point"; dout_width "Output width"
  dedispersor1 : Subsystem  mask{din_width=25, din_point=15, dout_width=25}
      mask prompts: din_width "Input width"; din_point "Input point"; dout_width "Output width"
  dedispersor10 : Subsystem  mask{din_width=25, din_point=15, dout_width=25}
      mask prompts: din_width "Input width"; din_point "Input point"; dout_width "Output width"
  dedispersor2 : Subsystem  mask{din_width=25, din_point=15, dout_width=25}
      mask prompts: din_width "Input width"; din_point "Input point"; dout_width "Output width"
  dedispersor3 : Subsystem  mask{din_width=25, din_point=15, dout_width=25}
      mask prompts: din_width "Input width"; din_point "Input point"; dout_width "Output width"
  dedispersor4 : Subsystem  mask{din_width=25, din_point=15, dout_width=25}
      mask prompts: din_width "Input width"; din_point "Input point"; dout_width "Output width"
  dedispersor5 : Subsystem  mask{din_width=25, din_point=15, dout_width=25}
      mask prompts: din_width "Input width"; din_point "Input point"; dout_width "Output width"
  dedispersor6 : Subsystem  mask{din_width=25, din_point=15, dout_width=25}
      mask prompts: din_width "Input width"; din_point "Input point"; dout_width "Output width"
  dedispersor7 : Subsystem  mask{din_width=25, din_point=15, dout_width=25}
      mask prompts: din_width "Input width"; din_point "Input point"; dout_width "Output width"
  dedispersor8 : Subsystem  mask{din_width=25, din_point=15, dout_width=25}
      mask prompts: din_width "Input width"; din_point "Input point"; dout_width "Output width"
  dedispersor9 : Subsystem  mask{din_width=25, din_point=15, dout_width=25}
      mask prompts: din_width "Input width"; din_point "Input point"; dout_width "Output width"
  delay_wideband_prog0 : Subsystem  AncestorBlock=casper_library_delays/delay_wideband_prog  mask(delay_wideband_prog){max_delay=128, n_inputs_bits=3, bram_latency=2, bram_type=Dual Port, async=off}
      mask prompts: max_delay "Max Delay (Sample Clks)"; n_inputs_bits "Number of Simultaneous Inputs(2^?)"; bram_latency "BRAM Latency"; bram_type "Select type of BRAM"; async "asynchronous operation"
      mask init:
      | delay_wideband_prog_init(gcb,...
      |     'max_delay',max_delay,...
      |     'n_inputs_bits',n_inputs_bits,...
      |     'bram_latency',bram_latency,...
      |     'bram_type',bram_type, ...
      |     'async', async);
      mask TypeOptions bram_type: Single Port | Dual Port
  enabled_vacc0 : Subsystem  mask{din_width=20, din_point=15, vec_len=64, dout_width=32}
      mask prompts: din_width "Input width"; din_point "Input point"; vec_len "vector length"; dout_width "Output width"
      mask help:
      | Enabled vector accumulator (the typical from casper is enabled in each clock
      | cycle).
  enabled_vacc1 : Subsystem  mask{din_width=20, din_point=15, vec_len=64, dout_width=32}
      mask prompts: din_width "Input width"; din_point "Input point"; vec_len "vector length"; dout_width "Output width"
      mask help:
      | Enabled vector accumulator (the typical from casper is enabled in each clock
      | cycle).
  enabled_vacc10 : Subsystem  mask{din_width=20, din_point=15, vec_len=64, dout_width=32}
      mask prompts: din_width "Input width"; din_point "Input point"; vec_len "vector length"; dout_width "Output width"
      mask help:
      | Enabled vector accumulator (the typical from casper is enabled in each clock
      | cycle).
  enabled_vacc2 : Subsystem  mask{din_width=20, din_point=15, vec_len=64, dout_width=32}
      mask prompts: din_width "Input width"; din_point "Input point"; vec_len "vector length"; dout_width "Output width"
      mask help:
      | Enabled vector accumulator (the typical from casper is enabled in each clock
      | cycle).
  enabled_vacc3 : Subsystem  mask{din_width=20, din_point=15, vec_len=64, dout_width=32}
      mask prompts: din_width "Input width"; din_point "Input point"; vec_len "vector length"; dout_width "Output width"
      mask help:
      | Enabled vector accumulator (the typical from casper is enabled in each clock
      | cycle).
  enabled_vacc4 : Subsystem  mask{din_width=20, din_point=15, vec_len=64, dout_width=32}
      mask prompts: din_width "Input width"; din_point "Input point"; vec_len "vector length"; dout_width "Output width"
      mask help:
      | Enabled vector accumulator (the typical from casper is enabled in each clock
      | cycle).
  enabled_vacc5 : Subsystem  mask{din_width=20, din_point=15, vec_len=64, dout_width=32}
      mask prompts: din_width "Input width"; din_point "Input point"; vec_len "vector length"; dout_width "Output width"
      mask help:
      | Enabled vector accumulator (the typical from casper is enabled in each clock
      | cycle).
  enabled_vacc6 : Subsystem  mask{din_width=20, din_point=15, vec_len=64, dout_width=32}
      mask prompts: din_width "Input width"; din_point "Input point"; vec_len "vector length"; dout_width "Output width"
      mask help:
      | Enabled vector accumulator (the typical from casper is enabled in each clock
      | cycle).
  enabled_vacc7 : Subsystem  mask{din_width=20, din_point=15, vec_len=64, dout_width=32}
      mask prompts: din_width "Input width"; din_point "Input point"; vec_len "vector length"; dout_width "Output width"
      mask help:
      | Enabled vector accumulator (the typical from casper is enabled in each clock
      | cycle).
  enabled_vacc8 : Subsystem  mask{din_width=20, din_point=15, vec_len=64, dout_width=32}
      mask prompts: din_width "Input width"; din_point "Input point"; vec_len "vector length"; dout_width "Output width"
      mask help:
      | Enabled vector accumulator (the typical from casper is enabled in each clock
      | cycle).
  enabled_vacc9 : Subsystem  mask{din_width=20, din_point=15, vec_len=64, dout_width=32}
      mask prompts: din_width "Input width"; din_point "Input point"; vec_len "vector length"; dout_width "Output width"
      mask help:
      | Enabled vector accumulator (the typical from casper is enabled in each clock
      | cycle).
  flag_convert : Subsystem  mask{shift_val=5, conv_width=18, conv_point=15}
      mask prompts: shift_val "shift"; conv_width "convert width"; conv_point "convert point"
  flag_power : Subsystem  mask{add_lat=5, mult_lat=3}
  m0_en1 : Subsystem
  m0_tree2 : Subsystem
  mov_avg0 : Subsystem  mask{din_width=25, din_point=15, win_size=128, dout_width=25}
      mask prompts: din_width "Input width"; din_point "Input point"; win_size "Avg window size"
  mov_avg1 : Subsystem  mask{din_width=25, din_point=15, win_size=128, dout_width=25}
      mask prompts: din_width "Input width"; din_point "Input point"; win_size "Avg window size"
  mov_avg10 : Subsystem  mask{din_width=25, din_point=15, win_size=128, dout_width=25}
      mask prompts: din_width "Input width"; din_point "Input point"; win_size "Avg window size"
  mov_avg2 : Subsystem  mask{din_width=25, din_point=15, win_size=128, dout_width=25}
      mask prompts: din_width "Input width"; din_point "Input point"; win_size "Avg window size"
  mov_avg3 : Subsystem  mask{din_width=25, din_point=15, win_size=128, dout_width=25}
      mask prompts: din_width "Input width"; din_point "Input point"; win_size "Avg window size"
  mov_avg4 : Subsystem  mask{din_width=25, din_point=15, win_size=128, dout_width=25}
      mask prompts: din_width "Input width"; din_point "Input point"; win_size "Avg window size"
  mov_avg5 : Subsystem  mask{din_width=25, din_point=15, win_size=128, dout_width=25}
      mask prompts: din_width "Input width"; din_point "Input point"; win_size "Avg window size"
  mov_avg6 : Subsystem  mask{din_width=25, din_point=15, win_size=128, dout_width=25}
      mask prompts: din_width "Input width"; din_point "Input point"; win_size "Avg window size"
  mov_avg7 : Subsystem  mask{din_width=25, din_point=15, win_size=128, dout_width=25}
      mask prompts: din_width "Input width"; din_point "Input point"; win_size "Avg window size"
  mov_avg8 : Subsystem  mask{din_width=25, din_point=15, win_size=128, dout_width=25}
      mask prompts: din_width "Input width"; din_point "Input point"; win_size "Avg window size"
  mov_avg9 : Subsystem  mask{din_width=25, din_point=15, win_size=128, dout_width=25}
      mask prompts: din_width "Input width"; din_point "Input point"; win_size "Avg window size"
  noise_diode : xps_library/gpio  Tag=xps:gpio  io_group=ROACH2:gpio  io_dir=out  arith_type=Boolean  bitwidth=1  bin_pt=0  bit_index=0  sample_period=512  use_single_ended=off  use_ddr=off  reg_iob=on  reg_clk_phase=0  termination=None
      link override convert: arith_type=Boolean  n_bits=1  bin_pt=0
  one_GbE : xps_library/one_GbE  Tag=xps:onegbe  local_en=off  dis_cpu_rx=on  dis_cpu_tx=off  cpu_promiscuous=off  local_mac=hex2dec('123456789abc')  local_ip=hex2dec('c0a8290a')  local_port=4321  local_gateway=1
  packetizer : Subsystem
  pcore : xps_library/pcore  Tag=xps:pcore  pcore_path=pfb_fft_8in_2048ch.ngc
  pipeline1 : Subsystem  AncestorBlock=casper_library_delays/pipeline  mask(pipeline){latency=1}
      mask help:
      | An explicitly laid-out delay line to avoid mapping to SRL16s
      | for use in pipelining to help achieve timing closure.
      mask init:
      | pipeline_init(gcb,'latency',latency);
      settings: AttributesFormatString=Latency = %<latency>
      mask Display:
      | port_label('input', 1, 'd');
      | port_label('output', 1, 'q');
      | disp(['Z^-', num2str(latency)]);
  pipeline10 : Subsystem  AncestorBlock=casper_library_delays/pipeline  mask(pipeline){latency=1}
      mask help:
      | An explicitly laid-out delay line to avoid mapping to SRL16s
      | for use in pipelining to help achieve timing closure.
      mask init:
      | pipeline_init(gcb,'latency',latency);
      settings: AttributesFormatString=Latency = %<latency>
      mask Display:
      | port_label('input', 1, 'd');
      | port_label('output', 1, 'q');
      | disp(['Z^-', num2str(latency)]);
  pipeline105 : Subsystem  AncestorBlock=casper_library_delays/pipeline  mask(pipeline){latency=3}
      mask help:
      | An explicitly laid-out delay line to avoid mapping to SRL16s
      | for use in pipelining to help achieve timing closure.
      mask init:
      | pipeline_init(gcb,'latency',latency);
      settings: AttributesFormatString=Latency = %<latency>
      mask Display:
      | port_label('input', 1, 'd');
      | port_label('output', 1, 'q');
      | disp(['Z^-', num2str(latency)]);
  pipeline106 : Subsystem  AncestorBlock=casper_library_delays/pipeline  mask(pipeline){latency=2}
      mask help:
      | An explicitly laid-out delay line to avoid mapping to SRL16s
      | for use in pipelining to help achieve timing closure.
      mask init:
      | pipeline_init(gcb,'latency',latency);
      settings: AttributesFormatString=Latency = %<latency>
      mask Display:
      | port_label('input', 1, 'd');
      | port_label('output', 1, 'q');
      | disp(['Z^-', num2str(latency)]);
  pipeline11 : Subsystem  AncestorBlock=casper_library_delays/pipeline  mask(pipeline){latency=1}
      mask help:
      | An explicitly laid-out delay line to avoid mapping to SRL16s
      | for use in pipelining to help achieve timing closure.
      mask init:
      | pipeline_init(gcb,'latency',latency);
      settings: AttributesFormatString=Latency = %<latency>
      mask Display:
      | port_label('input', 1, 'd');
      | port_label('output', 1, 'q');
      | disp(['Z^-', num2str(latency)]);
  pipeline12 : Subsystem  AncestorBlock=casper_library_delays/pipeline  mask(pipeline){latency=1}
      mask help:
      | An explicitly laid-out delay line to avoid mapping to SRL16s
      | for use in pipelining to help achieve timing closure.
      mask init:
      | pipeline_init(gcb,'latency',latency);
      settings: AttributesFormatString=Latency = %<latency>
      mask Display:
      | port_label('input', 1, 'd');
      | port_label('output', 1, 'q');
      | disp(['Z^-', num2str(latency)]);
  pipeline127 : Subsystem  AncestorBlock=casper_library_delays/pipeline  mask(pipeline){latency=2}
      mask help:
      | An explicitly laid-out delay line to avoid mapping to SRL16s
      | for use in pipelining to help achieve timing closure.
      mask init:
      | pipeline_init(gcb,'latency',latency);
      settings: AttributesFormatString=Latency = %<latency>
      mask Display:
      | port_label('input', 1, 'd');
      | port_label('output', 1, 'q');
      | disp(['Z^-', num2str(latency)]);
  pipeline14 : Subsystem  AncestorBlock=casper_library_delays/pipeline  mask(pipeline){latency=1}
      mask help:
      | An explicitly laid-out delay line to avoid mapping to SRL16s
      | for use in pipelining to help achieve timing closure.
      mask init:
      | pipeline_init(gcb,'latency',latency);
      settings: AttributesFormatString=Latency = %<latency>
      mask Display:
      | port_label('input', 1, 'd');
      | port_label('output', 1, 'q');
      | disp(['Z^-', num2str(latency)]);
  pipeline15 : Subsystem  AncestorBlock=casper_library_delays/pipeline  mask(pipeline){latency=1}
      mask help:
      | An explicitly laid-out delay line to avoid mapping to SRL16s
      | for use in pipelining to help achieve timing closure.
      mask init:
      | pipeline_init(gcb,'latency',latency);
      settings: AttributesFormatString=Latency = %<latency>
      mask Display:
      | port_label('input', 1, 'd');
      | port_label('output', 1, 'q');
      | disp(['Z^-', num2str(latency)]);
  pipeline16 : Subsystem  AncestorBlock=casper_library_delays/pipeline  mask(pipeline){latency=1}
      mask help:
      | An explicitly laid-out delay line to avoid mapping to SRL16s
      | for use in pipelining to help achieve timing closure.
      mask init:
      | pipeline_init(gcb,'latency',latency);
      settings: AttributesFormatString=Latency = %<latency>
      mask Display:
      | port_label('input', 1, 'd');
      | port_label('output', 1, 'q');
      | disp(['Z^-', num2str(latency)]);
  pipeline17 : Subsystem  AncestorBlock=casper_library_delays/pipeline  mask(pipeline){latency=2}
      mask help:
      | An explicitly laid-out delay line to avoid mapping to SRL16s
      | for use in pipelining to help achieve timing closure.
      mask init:
      | pipeline_init(gcb,'latency',latency);
      settings: AttributesFormatString=Latency = %<latency>
      mask Display:
      | port_label('input', 1, 'd');
      | port_label('output', 1, 'q');
      | disp(['Z^-', num2str(latency)]);
  pipeline18 : Subsystem  AncestorBlock=casper_library_delays/pipeline  mask(pipeline){latency=2}
      mask help:
      | An explicitly laid-out delay line to avoid mapping to SRL16s
      | for use in pipelining to help achieve timing closure.
      mask init:
      | pipeline_init(gcb,'latency',latency);
      settings: AttributesFormatString=Latency = %<latency>
      mask Display:
      | port_label('input', 1, 'd');
      | port_label('output', 1, 'q');
      | disp(['Z^-', num2str(latency)]);
  pipeline19 : Subsystem  AncestorBlock=casper_library_delays/pipeline  mask(pipeline){latency=2}
      mask help:
      | An explicitly laid-out delay line to avoid mapping to SRL16s
      | for use in pipelining to help achieve timing closure.
      mask init:
      | pipeline_init(gcb,'latency',latency);
      settings: AttributesFormatString=Latency = %<latency>
      mask Display:
      | port_label('input', 1, 'd');
      | port_label('output', 1, 'q');
      | disp(['Z^-', num2str(latency)]);
  pipeline2 : Subsystem  AncestorBlock=casper_library_delays/pipeline  mask(pipeline){latency=1}
      mask help:
      | An explicitly laid-out delay line to avoid mapping to SRL16s
      | for use in pipelining to help achieve timing closure.
      mask init:
      | pipeline_init(gcb,'latency',latency);
      settings: AttributesFormatString=Latency = %<latency>
      mask Display:
      | port_label('input', 1, 'd');
      | port_label('output', 1, 'q');
      | disp(['Z^-', num2str(latency)]);
  pipeline20 : Subsystem  AncestorBlock=casper_library_delays/pipeline  mask(pipeline){latency=2}
      mask help:
      | An explicitly laid-out delay line to avoid mapping to SRL16s
      | for use in pipelining to help achieve timing closure.
      mask init:
      | pipeline_init(gcb,'latency',latency);
      settings: AttributesFormatString=Latency = %<latency>
      mask Display:
      | port_label('input', 1, 'd');
      | port_label('output', 1, 'q');
      | disp(['Z^-', num2str(latency)]);
  pipeline21 : Subsystem  AncestorBlock=casper_library_delays/pipeline  mask(pipeline){latency=2}
      mask help:
      | An explicitly laid-out delay line to avoid mapping to SRL16s
      | for use in pipelining to help achieve timing closure.
      mask init:
      | pipeline_init(gcb,'latency',latency);
      settings: AttributesFormatString=Latency = %<latency>
      mask Display:
      | port_label('input', 1, 'd');
      | port_label('output', 1, 'q');
      | disp(['Z^-', num2str(latency)]);
  pipeline22 : Subsystem  AncestorBlock=casper_library_delays/pipeline  mask(pipeline){latency=2}
      mask help:
      | An explicitly laid-out delay line to avoid mapping to SRL16s
      | for use in pipelining to help achieve timing closure.
      mask init:
      | pipeline_init(gcb,'latency',latency);
      settings: AttributesFormatString=Latency = %<latency>
      mask Display:
      | port_label('input', 1, 'd');
      | port_label('output', 1, 'q');
      | disp(['Z^-', num2str(latency)]);
  pipeline23 : Subsystem  AncestorBlock=casper_library_delays/pipeline  mask(pipeline){latency=2}
      mask help:
      | An explicitly laid-out delay line to avoid mapping to SRL16s
      | for use in pipelining to help achieve timing closure.
      mask init:
      | pipeline_init(gcb,'latency',latency);
      settings: AttributesFormatString=Latency = %<latency>
      mask Display:
      | port_label('input', 1, 'd');
      | port_label('output', 1, 'q');
      | disp(['Z^-', num2str(latency)]);
  pipeline24 : Subsystem  AncestorBlock=casper_library_delays/pipeline  mask(pipeline){latency=2}
      mask help:
      | An explicitly laid-out delay line to avoid mapping to SRL16s
      | for use in pipelining to help achieve timing closure.
      mask init:
      | pipeline_init(gcb,'latency',latency);
      settings: AttributesFormatString=Latency = %<latency>
      mask Display:
      | port_label('input', 1, 'd');
      | port_label('output', 1, 'q');
      | disp(['Z^-', num2str(latency)]);
  pipeline26 : Subsystem  AncestorBlock=casper_library_delays/pipeline  mask(pipeline){latency=1}
      mask help:
      | An explicitly laid-out delay line to avoid mapping to SRL16s
      | for use in pipelining to help achieve timing closure.
      mask init:
      | pipeline_init(gcb,'latency',latency);
      settings: AttributesFormatString=Latency = %<latency>
      mask Display:
      | port_label('input', 1, 'd');
      | port_label('output', 1, 'q');
      | disp(['Z^-', num2str(latency)]);
  pipeline{27..30,39..42,46..47,53..54,61,66,69,74,96,276,298,403..405,407..409,421..424,428..430} (32 alike) : casper_library_delays/pipeline  latency=3
      settings: AttributesFormatString=Latency = %<latency>
  pipeline3 : Subsystem  AncestorBlock=casper_library_delays/pipeline  mask(pipeline){latency=1}
      mask help:
      | An explicitly laid-out delay line to avoid mapping to SRL16s
      | for use in pipelining to help achieve timing closure.
      mask init:
      | pipeline_init(gcb,'latency',latency);
      settings: AttributesFormatString=Latency = %<latency>
      mask Display:
      | port_label('input', 1, 'd');
      | port_label('output', 1, 'q');
      | disp(['Z^-', num2str(latency)]);
  pipeline31 : Subsystem  AncestorBlock=casper_library_delays/pipeline  mask(pipeline){latency=1}
      mask help:
      | An explicitly laid-out delay line to avoid mapping to SRL16s
      | for use in pipelining to help achieve timing closure.
      mask init:
      | pipeline_init(gcb,'latency',latency);
      settings: AttributesFormatString=Latency = %<latency>
      mask Display:
      | port_label('input', 1, 'd');
      | port_label('output', 1, 'q');
      | disp(['Z^-', num2str(latency)]);
  pipeline32 : Subsystem  AncestorBlock=casper_library_delays/pipeline  mask(pipeline){latency=1}
      mask help:
      | An explicitly laid-out delay line to avoid mapping to SRL16s
      | for use in pipelining to help achieve timing closure.
      mask init:
      | pipeline_init(gcb,'latency',latency);
      settings: AttributesFormatString=Latency = %<latency>
      mask Display:
      | port_label('input', 1, 'd');
      | port_label('output', 1, 'q');
      | disp(['Z^-', num2str(latency)]);
  pipeline33 : Subsystem  AncestorBlock=casper_library_delays/pipeline  mask(pipeline){latency=1}
      mask help:
      | An explicitly laid-out delay line to avoid mapping to SRL16s
      | for use in pipelining to help achieve timing closure.
      mask init:
      | pipeline_init(gcb,'latency',latency);
      settings: AttributesFormatString=Latency = %<latency>
      mask Display:
      | port_label('input', 1, 'd');
      | port_label('output', 1, 'q');
      | disp(['Z^-', num2str(latency)]);
  pipeline34 : Subsystem  AncestorBlock=casper_library_delays/pipeline  mask(pipeline){latency=1}
      mask help:
      | An explicitly laid-out delay line to avoid mapping to SRL16s
      | for use in pipelining to help achieve timing closure.
      mask init:
      | pipeline_init(gcb,'latency',latency);
      settings: AttributesFormatString=Latency = %<latency>
      mask Display:
      | port_label('input', 1, 'd');
      | port_label('output', 1, 'q');
      | disp(['Z^-', num2str(latency)]);
  pipeline35 : Subsystem  AncestorBlock=casper_library_delays/pipeline  mask(pipeline){latency=1}
      mask help:
      | An explicitly laid-out delay line to avoid mapping to SRL16s
      | for use in pipelining to help achieve timing closure.
      mask init:
      | pipeline_init(gcb,'latency',latency);
      settings: AttributesFormatString=Latency = %<latency>
      mask Display:
      | port_label('input', 1, 'd');
      | port_label('output', 1, 'q');
      | disp(['Z^-', num2str(latency)]);
  pipeline36 : Subsystem  AncestorBlock=casper_library_delays/pipeline  mask(pipeline){latency=1}
      mask help:
      | An explicitly laid-out delay line to avoid mapping to SRL16s
      | for use in pipelining to help achieve timing closure.
      mask init:
      | pipeline_init(gcb,'latency',latency);
      settings: AttributesFormatString=Latency = %<latency>
      mask Display:
      | port_label('input', 1, 'd');
      | port_label('output', 1, 'q');
      | disp(['Z^-', num2str(latency)]);
  pipeline37 : Subsystem  AncestorBlock=casper_library_delays/pipeline  mask(pipeline){latency=1}
      mask help:
      | An explicitly laid-out delay line to avoid mapping to SRL16s
      | for use in pipelining to help achieve timing closure.
      mask init:
      | pipeline_init(gcb,'latency',latency);
      settings: AttributesFormatString=Latency = %<latency>
      mask Display:
      | port_label('input', 1, 'd');
      | port_label('output', 1, 'q');
      | disp(['Z^-', num2str(latency)]);
  pipeline38 : Subsystem  AncestorBlock=casper_library_delays/pipeline  mask(pipeline){latency=1}
      mask help:
      | An explicitly laid-out delay line to avoid mapping to SRL16s
      | for use in pipelining to help achieve timing closure.
      mask init:
      | pipeline_init(gcb,'latency',latency);
      settings: AttributesFormatString=Latency = %<latency>
      mask Display:
      | port_label('input', 1, 'd');
      | port_label('output', 1, 'q');
      | disp(['Z^-', num2str(latency)]);
  pipeline406 : Subsystem  AncestorBlock=casper_library_delays/pipeline  mask(pipeline){latency=5}
      mask help:
      | An explicitly laid-out delay line to avoid mapping to SRL16s
      | for use in pipelining to help achieve timing closure.
      mask init:
      | pipeline_init(gcb,'latency',latency);
      settings: AttributesFormatString=Latency = %<latency>
      mask Display:
      | port_label('input', 1, 'd');
      | port_label('output', 1, 'q');
      | disp(['Z^-', num2str(latency)]);
  pipeline43 : Subsystem  AncestorBlock=casper_library_delays/pipeline  mask(pipeline){latency=1}
      mask help:
      | An explicitly laid-out delay line to avoid mapping to SRL16s
      | for use in pipelining to help achieve timing closure.
      mask init:
      | pipeline_init(gcb,'latency',latency);
      settings: AttributesFormatString=Latency = %<latency>
      mask Display:
      | port_label('input', 1, 'd');
      | port_label('output', 1, 'q');
      | disp(['Z^-', num2str(latency)]);
  pipeline45 : Subsystem  AncestorBlock=casper_library_delays/pipeline  mask(pipeline){latency=1}
      mask help:
      | An explicitly laid-out delay line to avoid mapping to SRL16s
      | for use in pipelining to help achieve timing closure.
      mask init:
      | pipeline_init(gcb,'latency',latency);
      settings: AttributesFormatString=Latency = %<latency>
      mask Display:
      | port_label('input', 1, 'd');
      | port_label('output', 1, 'q');
      | disp(['Z^-', num2str(latency)]);
  pipeline48 : Subsystem  AncestorBlock=casper_library_delays/pipeline  mask(pipeline){latency=1}
      mask help:
      | An explicitly laid-out delay line to avoid mapping to SRL16s
      | for use in pipelining to help achieve timing closure.
      mask init:
      | pipeline_init(gcb,'latency',latency);
      settings: AttributesFormatString=Latency = %<latency>
      mask Display:
      | port_label('input', 1, 'd');
      | port_label('output', 1, 'q');
      | disp(['Z^-', num2str(latency)]);
  pipeline5 : Subsystem  AncestorBlock=casper_library_delays/pipeline  mask(pipeline){latency=1}
      mask help:
      | An explicitly laid-out delay line to avoid mapping to SRL16s
      | for use in pipelining to help achieve timing closure.
      mask init:
      | pipeline_init(gcb,'latency',latency);
      settings: AttributesFormatString=Latency = %<latency>
      mask Display:
      | port_label('input', 1, 'd');
      | port_label('output', 1, 'q');
      | disp(['Z^-', num2str(latency)]);
  pipeline51 : Subsystem  AncestorBlock=casper_library_delays/pipeline  mask(pipeline){latency=1}
      mask help:
      | An explicitly laid-out delay line to avoid mapping to SRL16s
      | for use in pipelining to help achieve timing closure.
      mask init:
      | pipeline_init(gcb,'latency',latency);
      settings: AttributesFormatString=Latency = %<latency>
      mask Display:
      | port_label('input', 1, 'd');
      | port_label('output', 1, 'q');
      | disp(['Z^-', num2str(latency)]);
  pipeline56 : Subsystem  AncestorBlock=casper_library_delays/pipeline  mask(pipeline){latency=1}
      mask help:
      | An explicitly laid-out delay line to avoid mapping to SRL16s
      | for use in pipelining to help achieve timing closure.
      mask init:
      | pipeline_init(gcb,'latency',latency);
      settings: AttributesFormatString=Latency = %<latency>
      mask Display:
      | port_label('input', 1, 'd');
      | port_label('output', 1, 'q');
      | disp(['Z^-', num2str(latency)]);
  pipeline57 : Subsystem  AncestorBlock=casper_library_delays/pipeline  mask(pipeline){latency=1}
      mask help:
      | An explicitly laid-out delay line to avoid mapping to SRL16s
      | for use in pipelining to help achieve timing closure.
      mask init:
      | pipeline_init(gcb,'latency',latency);
      settings: AttributesFormatString=Latency = %<latency>
      mask Display:
      | port_label('input', 1, 'd');
      | port_label('output', 1, 'q');
      | disp(['Z^-', num2str(latency)]);
  pipeline58 : Subsystem  AncestorBlock=casper_library_delays/pipeline  mask(pipeline){latency=1}
      mask help:
      | An explicitly laid-out delay line to avoid mapping to SRL16s
      | for use in pipelining to help achieve timing closure.
      mask init:
      | pipeline_init(gcb,'latency',latency);
      settings: AttributesFormatString=Latency = %<latency>
      mask Display:
      | port_label('input', 1, 'd');
      | port_label('output', 1, 'q');
      | disp(['Z^-', num2str(latency)]);
  pipeline59 : Subsystem  AncestorBlock=casper_library_delays/pipeline  mask(pipeline){latency=1}
      mask help:
      | An explicitly laid-out delay line to avoid mapping to SRL16s
      | for use in pipelining to help achieve timing closure.
      mask init:
      | pipeline_init(gcb,'latency',latency);
      settings: AttributesFormatString=Latency = %<latency>
      mask Display:
      | port_label('input', 1, 'd');
      | port_label('output', 1, 'q');
      | disp(['Z^-', num2str(latency)]);
  pipeline60 : Subsystem  AncestorBlock=casper_library_delays/pipeline  mask(pipeline){latency=1}
      mask help:
      | An explicitly laid-out delay line to avoid mapping to SRL16s
      | for use in pipelining to help achieve timing closure.
      mask init:
      | pipeline_init(gcb,'latency',latency);
      settings: AttributesFormatString=Latency = %<latency>
      mask Display:
      | port_label('input', 1, 'd');
      | port_label('output', 1, 'q');
      | disp(['Z^-', num2str(latency)]);
  pipeline62 : Subsystem  AncestorBlock=casper_library_delays/pipeline  mask(pipeline){latency=1}
      mask help:
      | An explicitly laid-out delay line to avoid mapping to SRL16s
      | for use in pipelining to help achieve timing closure.
      mask init:
      | pipeline_init(gcb,'latency',latency);
      settings: AttributesFormatString=Latency = %<latency>
      mask Display:
      | port_label('input', 1, 'd');
      | port_label('output', 1, 'q');
      | disp(['Z^-', num2str(latency)]);
  pipeline63 : Subsystem  AncestorBlock=casper_library_delays/pipeline  mask(pipeline){latency=1}
      mask help:
      | An explicitly laid-out delay line to avoid mapping to SRL16s
      | for use in pipelining to help achieve timing closure.
      mask init:
      | pipeline_init(gcb,'latency',latency);
      settings: AttributesFormatString=Latency = %<latency>
      mask Display:
      | port_label('input', 1, 'd');
      | port_label('output', 1, 'q');
      | disp(['Z^-', num2str(latency)]);
  pipeline64 : Subsystem  AncestorBlock=casper_library_delays/pipeline  mask(pipeline){latency=1}
      mask help:
      | An explicitly laid-out delay line to avoid mapping to SRL16s
      | for use in pipelining to help achieve timing closure.
      mask init:
      | pipeline_init(gcb,'latency',latency);
      settings: AttributesFormatString=Latency = %<latency>
      mask Display:
      | port_label('input', 1, 'd');
      | port_label('output', 1, 'q');
      | disp(['Z^-', num2str(latency)]);
  pipeline65 : Subsystem  AncestorBlock=casper_library_delays/pipeline  mask(pipeline){latency=1}
      mask help:
      | An explicitly laid-out delay line to avoid mapping to SRL16s
      | for use in pipelining to help achieve timing closure.
      mask init:
      | pipeline_init(gcb,'latency',latency);
      settings: AttributesFormatString=Latency = %<latency>
      mask Display:
      | port_label('input', 1, 'd');
      | port_label('output', 1, 'q');
      | disp(['Z^-', num2str(latency)]);
  pipeline67 : Subsystem  AncestorBlock=casper_library_delays/pipeline  mask(pipeline){latency=1}
      mask help:
      | An explicitly laid-out delay line to avoid mapping to SRL16s
      | for use in pipelining to help achieve timing closure.
      mask init:
      | pipeline_init(gcb,'latency',latency);
      settings: AttributesFormatString=Latency = %<latency>
      mask Display:
      | port_label('input', 1, 'd');
      | port_label('output', 1, 'q');
      | disp(['Z^-', num2str(latency)]);
  pipeline68 : Subsystem  AncestorBlock=casper_library_delays/pipeline  mask(pipeline){latency=1}
      mask help:
      | An explicitly laid-out delay line to avoid mapping to SRL16s
      | for use in pipelining to help achieve timing closure.
      mask init:
      | pipeline_init(gcb,'latency',latency);
      settings: AttributesFormatString=Latency = %<latency>
      mask Display:
      | port_label('input', 1, 'd');
      | port_label('output', 1, 'q');
      | disp(['Z^-', num2str(latency)]);
  pipeline7 : Subsystem  AncestorBlock=casper_library_delays/pipeline  mask(pipeline){latency=1}
      mask help:
      | An explicitly laid-out delay line to avoid mapping to SRL16s
      | for use in pipelining to help achieve timing closure.
      mask init:
      | pipeline_init(gcb,'latency',latency);
      settings: AttributesFormatString=Latency = %<latency>
      mask Display:
      | port_label('input', 1, 'd');
      | port_label('output', 1, 'q');
      | disp(['Z^-', num2str(latency)]);
  pipeline70 : Subsystem  AncestorBlock=casper_library_delays/pipeline  mask(pipeline){latency=1}
      mask help:
      | An explicitly laid-out delay line to avoid mapping to SRL16s
      | for use in pipelining to help achieve timing closure.
      mask init:
      | pipeline_init(gcb,'latency',latency);
      settings: AttributesFormatString=Latency = %<latency>
      mask Display:
      | port_label('input', 1, 'd');
      | port_label('output', 1, 'q');
      | disp(['Z^-', num2str(latency)]);
  pipeline71 : Subsystem  AncestorBlock=casper_library_delays/pipeline  mask(pipeline){latency=1}
      mask help:
      | An explicitly laid-out delay line to avoid mapping to SRL16s
      | for use in pipelining to help achieve timing closure.
      mask init:
      | pipeline_init(gcb,'latency',latency);
      settings: AttributesFormatString=Latency = %<latency>
      mask Display:
      | port_label('input', 1, 'd');
      | port_label('output', 1, 'q');
      | disp(['Z^-', num2str(latency)]);
  pipeline72 : Subsystem  AncestorBlock=casper_library_delays/pipeline  mask(pipeline){latency=1}
      mask help:
      | An explicitly laid-out delay line to avoid mapping to SRL16s
      | for use in pipelining to help achieve timing closure.
      mask init:
      | pipeline_init(gcb,'latency',latency);
      settings: AttributesFormatString=Latency = %<latency>
      mask Display:
      | port_label('input', 1, 'd');
      | port_label('output', 1, 'q');
      | disp(['Z^-', num2str(latency)]);
  pipeline73 : Subsystem  AncestorBlock=casper_library_delays/pipeline  mask(pipeline){latency=1}
      mask help:
      | An explicitly laid-out delay line to avoid mapping to SRL16s
      | for use in pipelining to help achieve timing closure.
      mask init:
      | pipeline_init(gcb,'latency',latency);
      settings: AttributesFormatString=Latency = %<latency>
      mask Display:
      | port_label('input', 1, 'd');
      | port_label('output', 1, 'q');
      | disp(['Z^-', num2str(latency)]);
  pipeline75 : Subsystem  AncestorBlock=casper_library_delays/pipeline  mask(pipeline){latency=2}
      mask help:
      | An explicitly laid-out delay line to avoid mapping to SRL16s
      | for use in pipelining to help achieve timing closure.
      mask init:
      | pipeline_init(gcb,'latency',latency);
      settings: AttributesFormatString=Latency = %<latency>
      mask Display:
      | port_label('input', 1, 'd');
      | port_label('output', 1, 'q');
      | disp(['Z^-', num2str(latency)]);
  pipeline79 : Subsystem  AncestorBlock=casper_library_delays/pipeline  mask(pipeline){latency=2}
      mask help:
      | An explicitly laid-out delay line to avoid mapping to SRL16s
      | for use in pipelining to help achieve timing closure.
      mask init:
      | pipeline_init(gcb,'latency',latency);
      settings: AttributesFormatString=Latency = %<latency>
      mask Display:
      | port_label('input', 1, 'd');
      | port_label('output', 1, 'q');
      | disp(['Z^-', num2str(latency)]);
  pipeline8 : Subsystem  AncestorBlock=casper_library_delays/pipeline  mask(pipeline){latency=1}
      mask help:
      | An explicitly laid-out delay line to avoid mapping to SRL16s
      | for use in pipelining to help achieve timing closure.
      mask init:
      | pipeline_init(gcb,'latency',latency);
      settings: AttributesFormatString=Latency = %<latency>
      mask Display:
      | port_label('input', 1, 'd');
      | port_label('output', 1, 'q');
      | disp(['Z^-', num2str(latency)]);
  pipeline80 : Subsystem  AncestorBlock=casper_library_delays/pipeline  mask(pipeline){latency=2}
      mask help:
      | An explicitly laid-out delay line to avoid mapping to SRL16s
      | for use in pipelining to help achieve timing closure.
      mask init:
      | pipeline_init(gcb,'latency',latency);
      settings: AttributesFormatString=Latency = %<latency>
      mask Display:
      | port_label('input', 1, 'd');
      | port_label('output', 1, 'q');
      | disp(['Z^-', num2str(latency)]);
  pipeline83 : Subsystem  AncestorBlock=casper_library_delays/pipeline  mask(pipeline){latency=2}
      mask help:
      | An explicitly laid-out delay line to avoid mapping to SRL16s
      | for use in pipelining to help achieve timing closure.
      mask init:
      | pipeline_init(gcb,'latency',latency);
      settings: AttributesFormatString=Latency = %<latency>
      mask Display:
      | port_label('input', 1, 'd');
      | port_label('output', 1, 'q');
      | disp(['Z^-', num2str(latency)]);
  pipeline84 : Subsystem  AncestorBlock=casper_library_delays/pipeline  mask(pipeline){latency=2}
      mask help:
      | An explicitly laid-out delay line to avoid mapping to SRL16s
      | for use in pipelining to help achieve timing closure.
      mask init:
      | pipeline_init(gcb,'latency',latency);
      settings: AttributesFormatString=Latency = %<latency>
      mask Display:
      | port_label('input', 1, 'd');
      | port_label('output', 1, 'q');
      | disp(['Z^-', num2str(latency)]);
  pipeline87 : Subsystem  AncestorBlock=casper_library_delays/pipeline  mask(pipeline){latency=2}
      mask help:
      | An explicitly laid-out delay line to avoid mapping to SRL16s
      | for use in pipelining to help achieve timing closure.
      mask init:
      | pipeline_init(gcb,'latency',latency);
      settings: AttributesFormatString=Latency = %<latency>
      mask Display:
      | port_label('input', 1, 'd');
      | port_label('output', 1, 'q');
      | disp(['Z^-', num2str(latency)]);
  pipeline88 : Subsystem  AncestorBlock=casper_library_delays/pipeline  mask(pipeline){latency=2}
      mask help:
      | An explicitly laid-out delay line to avoid mapping to SRL16s
      | for use in pipelining to help achieve timing closure.
      mask init:
      | pipeline_init(gcb,'latency',latency);
      settings: AttributesFormatString=Latency = %<latency>
      mask Display:
      | port_label('input', 1, 'd');
      | port_label('output', 1, 'q');
      | disp(['Z^-', num2str(latency)]);
  pipeline9 : Subsystem  AncestorBlock=casper_library_delays/pipeline  mask(pipeline){latency=1}
      mask help:
      | An explicitly laid-out delay line to avoid mapping to SRL16s
      | for use in pipelining to help achieve timing closure.
      mask init:
      | pipeline_init(gcb,'latency',latency);
      settings: AttributesFormatString=Latency = %<latency>
      mask Display:
      | port_label('input', 1, 'd');
      | port_label('output', 1, 'q');
      | disp(['Z^-', num2str(latency)]);
  pipeline90 : Subsystem  AncestorBlock=casper_library_delays/pipeline  mask(pipeline){latency=2}
      mask help:
      | An explicitly laid-out delay line to avoid mapping to SRL16s
      | for use in pipelining to help achieve timing closure.
      mask init:
      | pipeline_init(gcb,'latency',latency);
      settings: AttributesFormatString=Latency = %<latency>
      mask Display:
      | port_label('input', 1, 'd');
      | port_label('output', 1, 'q');
      | disp(['Z^-', num2str(latency)]);
  pipeline92 : Subsystem  AncestorBlock=casper_library_delays/pipeline  mask(pipeline){latency=2}
      mask help:
      | An explicitly laid-out delay line to avoid mapping to SRL16s
      | for use in pipelining to help achieve timing closure.
      mask init:
      | pipeline_init(gcb,'latency',latency);
      settings: AttributesFormatString=Latency = %<latency>
      mask Display:
      | port_label('input', 1, 'd');
      | port_label('output', 1, 'q');
      | disp(['Z^-', num2str(latency)]);
  pipeline93 : Subsystem  AncestorBlock=casper_library_delays/pipeline  mask(pipeline){latency=2}
      mask help:
      | An explicitly laid-out delay line to avoid mapping to SRL16s
      | for use in pipelining to help achieve timing closure.
      mask init:
      | pipeline_init(gcb,'latency',latency);
      settings: AttributesFormatString=Latency = %<latency>
      mask Display:
      | port_label('input', 1, 'd');
      | port_label('output', 1, 'q');
      | disp(['Z^-', num2str(latency)]);
  pipeline95 : Subsystem  AncestorBlock=casper_library_delays/pipeline  mask(pipeline){latency=2}
      mask help:
      | An explicitly laid-out delay line to avoid mapping to SRL16s
      | for use in pipelining to help achieve timing closure.
      mask init:
      | pipeline_init(gcb,'latency',latency);
      settings: AttributesFormatString=Latency = %<latency>
      mask Display:
      | port_label('input', 1, 'd');
      | port_label('output', 1, 'q');
      | disp(['Z^-', num2str(latency)]);
  pipeline99 : Subsystem  AncestorBlock=casper_library_delays/pipeline  mask(pipeline){latency=2}
      mask help:
      | An explicitly laid-out delay line to avoid mapping to SRL16s
      | for use in pipelining to help achieve timing closure.
      mask init:
      | pipeline_init(gcb,'latency',latency);
      settings: AttributesFormatString=Latency = %<latency>
      mask Display:
      | port_label('input', 1, 'd');
      | port_label('output', 1, 'q');
      | disp(['Z^-', num2str(latency)]);
  post_dedisp_conv0 : Subsystem  mask{shift_val=0, conv_width=25, conv_point=15}
      mask prompts: shift_val "shift"; conv_width "convert width"; conv_point "convert point"
  post_dedisp_conv1 : Subsystem  mask{shift_val=0, conv_width=25, conv_point=15}
      mask prompts: shift_val "shift"; conv_width "convert width"; conv_point "convert point"
  post_dedisp_conv10 : Subsystem  mask{shift_val=0, conv_width=25, conv_point=15}
      mask prompts: shift_val "shift"; conv_width "convert width"; conv_point "convert point"
  post_dedisp_conv2 : Subsystem  mask{shift_val=0, conv_width=25, conv_point=15}
      mask prompts: shift_val "shift"; conv_width "convert width"; conv_point "convert point"
  post_dedisp_conv3 : Subsystem  mask{shift_val=0, conv_width=25, conv_point=15}
      mask prompts: shift_val "shift"; conv_width "convert width"; conv_point "convert point"
  post_dedisp_conv4 : Subsystem  mask{shift_val=0, conv_width=25, conv_point=15}
      mask prompts: shift_val "shift"; conv_width "convert width"; conv_point "convert point"
  post_dedisp_conv5 : Subsystem  mask{shift_val=0, conv_width=25, conv_point=15}
      mask prompts: shift_val "shift"; conv_width "convert width"; conv_point "convert point"
  post_dedisp_conv6 : Subsystem  mask{shift_val=0, conv_width=25, conv_point=15}
      mask prompts: shift_val "shift"; conv_width "convert width"; conv_point "convert point"
  post_dedisp_conv7 : Subsystem  mask{shift_val=0, conv_width=25, conv_point=15}
      mask prompts: shift_val "shift"; conv_width "convert width"; conv_point "convert point"
  post_dedisp_conv8 : Subsystem  mask{shift_val=0, conv_width=25, conv_point=15}
      mask prompts: shift_val "shift"; conv_width "convert width"; conv_point "convert point"
  post_dedisp_conv9 : Subsystem  mask{shift_val=0, conv_width=25, conv_point=15}
      mask prompts: shift_val "shift"; conv_width "convert width"; conv_point "convert point"
  post_dedisp_delay0 : Subsystem  mask{lat=1}
  post_dedisp_delay1 : Subsystem  mask{lat=1}
  post_dedisp_delay10 : Subsystem  mask{lat=1}
  post_dedisp_delay2 : Subsystem  mask{lat=1}
  post_dedisp_delay3 : Subsystem  mask{lat=1}
  post_dedisp_delay4 : Subsystem  mask{lat=1}
  post_dedisp_delay5 : Subsystem  mask{lat=1}
  post_dedisp_delay6 : Subsystem  mask{lat=1}
  post_dedisp_delay7 : Subsystem  mask{lat=1}
  post_dedisp_delay8 : Subsystem  mask{lat=1}
  post_dedisp_delay9 : Subsystem  mask{lat=1}
  post_fft_delay0 : Subsystem  mask{lat=3}
  post_flag_delay : Subsystem  mask{lat=3}
  post_flag_delay1 : Subsystem  mask{lat=2}
  power_convert0 : Subsystem  mask{shift_val=13, conv_width=20, conv_point=19}
      mask prompts: shift_val "shift"; conv_width "convert width"; conv_point "convert point"
  pre_bram_delay0 : Subsystem  mask{lat=2}
  pre_dedisp_acc_conv : Subsystem  mask{shift_val=0, conv_width=20, conv_point=15}
      mask prompts: shift_val "shift"; conv_width "convert width"; conv_point "convert point"
  pre_dedisp_conv0 : Subsystem  mask{shift_val=0, conv_width=25, conv_point=15}
      mask prompts: shift_val "shift"; conv_width "convert width"; conv_point "convert point"
  pre_dedisp_conv1 : Subsystem  mask{shift_val=0, conv_width=25, conv_point=15}
      mask prompts: shift_val "shift"; conv_width "convert width"; conv_point "convert point"
  pre_dedisp_conv10 : Subsystem  mask{shift_val=0, conv_width=25, conv_point=15}
      mask prompts: shift_val "shift"; conv_width "convert width"; conv_point "convert point"
  pre_dedisp_conv2 : Subsystem  mask{shift_val=0, conv_width=25, conv_point=15}
      mask prompts: shift_val "shift"; conv_width "convert width"; conv_point "convert point"
  pre_dedisp_conv3 : Subsystem  mask{shift_val=0, conv_width=25, conv_point=15}
      mask prompts: shift_val "shift"; conv_width "convert width"; conv_point "convert point"
  pre_dedisp_conv4 : Subsystem  mask{shift_val=0, conv_width=25, conv_point=15}
      mask prompts: shift_val "shift"; conv_width "convert width"; conv_point "convert point"
  pre_dedisp_conv5 : Subsystem  mask{shift_val=0, conv_width=25, conv_point=15}
      mask prompts: shift_val "shift"; conv_width "convert width"; conv_point "convert point"
  pre_dedisp_conv6 : Subsystem  mask{shift_val=0, conv_width=25, conv_point=15}
      mask prompts: shift_val "shift"; conv_width "convert width"; conv_point "convert point"
  pre_dedisp_conv7 : Subsystem  mask{shift_val=0, conv_width=25, conv_point=15}
      mask prompts: shift_val "shift"; conv_width "convert width"; conv_point "convert point"
  pre_dedisp_conv8 : Subsystem  mask{shift_val=0, conv_width=25, conv_point=15}
      mask prompts: shift_val "shift"; conv_width "convert width"; conv_point "convert point"
  pre_dedisp_conv9 : Subsystem  mask{shift_val=0, conv_width=25, conv_point=15}
      mask prompts: shift_val "shift"; conv_width "convert width"; conv_point "convert point"
  pre_dedisp_delay0 : Subsystem  mask{lat=2}
  pre_dedisp_delay1 : Subsystem  mask{lat=2}
  pre_dedisp_delay10 : Subsystem  mask{lat=2}
  pre_dedisp_delay2 : Subsystem  mask{lat=2}
  pre_dedisp_delay3 : Subsystem  mask{lat=2}
  pre_dedisp_delay4 : Subsystem  mask{lat=2}
  pre_dedisp_delay5 : Subsystem  mask{lat=2}
  pre_dedisp_delay6 : Subsystem  mask{lat=2}
  pre_dedisp_delay7 : Subsystem  mask{lat=2}
  pre_dedisp_delay8 : Subsystem  mask{lat=2}
  pre_dedisp_delay9 : Subsystem  mask{lat=2}
  pre_pfb_delay1 : Subsystem  mask{lat=2}
  ring : Subsystem
  simple_bram_vacc_0_0 : Subsystem  AncestorBlock=casper_library_accumulators/simple_bram_vacc  mask(simple_bram_vacc){vec_len=512, arith_type=Unsigned, n_bits=32, bin_pt=19}
      mask prompts: vec_len "Vector length:"; arith_type "Output type:"; n_bits "Bit width (output):"; bin_pt "Binary point (output):"
      mask help: This simple vector accumulator is based on a shift register. It outputs its previous accumulated vector after a new_acc pulse is received.
      mask init:
      | simple_bram_vacc_init(gcb, ...
      |     'vec_len', vec_len, ...
      |     'arith_type', arith_type, ...
      |     'n_bits', n_bits, ...
      |     'bin_pt', bin_pt);
      mask TypeOptions arith_type: Signed | Unsigned
  simple_bram_vacc_0_1 : Subsystem  AncestorBlock=casper_library_accumulators/simple_bram_vacc  mask(simple_bram_vacc){vec_len=512, arith_type=Unsigned, n_bits=32, bin_pt=19}
      mask prompts: vec_len "Vector length:"; arith_type "Output type:"; n_bits "Bit width (output):"; bin_pt "Binary point (output):"
      mask help: This simple vector accumulator is based on a shift register. It outputs its previous accumulated vector after a new_acc pulse is received.
      mask init:
      | simple_bram_vacc_init(gcb, ...
      |     'vec_len', vec_len, ...
      |     'arith_type', arith_type, ...
      |     'n_bits', n_bits, ...
      |     'bin_pt', bin_pt);
      mask TypeOptions arith_type: Signed | Unsigned
  simple_bram_vacc_0_2 : Subsystem  AncestorBlock=casper_library_accumulators/simple_bram_vacc  mask(simple_bram_vacc){vec_len=512, arith_type=Unsigned, n_bits=32, bin_pt=19}
      mask prompts: vec_len "Vector length:"; arith_type "Output type:"; n_bits "Bit width (output):"; bin_pt "Binary point (output):"
      mask help: This simple vector accumulator is based on a shift register. It outputs its previous accumulated vector after a new_acc pulse is received.
      mask init:
      | simple_bram_vacc_init(gcb, ...
      |     'vec_len', vec_len, ...
      |     'arith_type', arith_type, ...
      |     'n_bits', n_bits, ...
      |     'bin_pt', bin_pt);
      mask TypeOptions arith_type: Signed | Unsigned
  simple_bram_vacc_0_3 : Subsystem  AncestorBlock=casper_library_accumulators/simple_bram_vacc  mask(simple_bram_vacc){vec_len=512, arith_type=Unsigned, n_bits=32, bin_pt=19}
      mask prompts: vec_len "Vector length:"; arith_type "Output type:"; n_bits "Bit width (output):"; bin_pt "Binary point (output):"
      mask help: This simple vector accumulator is based on a shift register. It outputs its previous accumulated vector after a new_acc pulse is received.
      mask init:
      | simple_bram_vacc_init(gcb, ...
      |     'vec_len', vec_len, ...
      |     'arith_type', arith_type, ...
      |     'n_bits', n_bits, ...
      |     'bin_pt', bin_pt);
      mask TypeOptions arith_type: Signed | Unsigned
  snapshot : Subsystem  Tag=casper:snapshot  AncestorBlock=casper_library_scopes/snapshot  mask(snapshot){storage=bram, dram_dimm=1, dram_clock=200, nsamples=10, data_width=64, offset=off, circap=off, value=off, use_dsp48=off}
      mask prompts: storage "Storage medium"; dram_dimm "DRAM dimm"; dram_clock "DRAM clock rate"; nsamples "Number of Samples (2^?)"; data_width "Data width"; offset "Start delay support"; circap "Circular capture support"; value "Extra value capture support"; use_dsp48 "Use DSP48s to implement counters"
      mask help:
      | Standard snap block, but with the following optional extras;
      |  1) Optionally delay the fabric trigger by a user-specified number of valids.
      |  2) Capture continuously after a trigger until a stop pulse is received. Data is captured into BRAM continuously, with old data being overwritten until a stop command is received. Then stop capturing when memory is filled. This enables you to get some data before and some data after the stop pulse. Use the 'tr_en_cnt' register to determine where you are in your vector. 'Addr' register's MSb now indicates 'busy capturing'.
      |  3) Optionally capture a value on an input port to a register at the same time as the first data sample.
      |  4) Implement counters using DSP48Es to save resources.
      mask init: same as arte/adcsnap0
      mask TypeOptions storage: bram | dram
      mask Callback storage: snapshot_callback();
      mask TypeOptions dram_dimm: 1 | 2 | 3 | 4
      mask TypeOptions dram_clock: 200 | 250 | 266 | 300 | 333
      mask TypeOptions data_width: 8 | 16 | 32 | 64 | 128
  sync_gen : Subsystem  AncestorBlock=casper_library_misc/sync_gen  mask(sync_gen){sim_acc_len=1, fft_size=4096, fft_simult_inputs=8, pfb_fir_taps=3, reorder_vec=[2,2,9], scale=1}
      mask prompts: sim_acc_len "Simulation Accumulation Length"; fft_size "FFT Size"; fft_simult_inputs "Simultaneous Inputs (FFT)"; pfb_fir_taps "Taps in pfb_fir (use 1 if no pfb_fir)"; reorder_vec "Reorder Orders (e.g. [2 2 2])"
      mask help:
      | This block computes the sync period based on system parameters as
      | described in Casper memo.  Detailed descritions of the block's
      | variables can be found in the 'Block Documentation' section of
      | the CASPER wiki.
      mask init:
      | sync_gen_init(gcb, ...
      |     'sim_acc_len', sim_acc_len, ...
      |     'fft_size', fft_size, ...
      |     'fft_simult_inputs', fft_simult_inputs,...
      |     'pfb_fir_taps', pfb_fir_taps, ...
      |     'reorder_vec', reorder_vec, ...
      |     'scale', scale);
      settings: AttributesFormatString=sim_sync_period=27648
      mask Help:
      | SyncPeriod=LCM(reorder_vec)*(acc_num)*(pfb_fir_len)*(fft_size/fft_simult_inputs)
      | 
      | See CASPER sync pulse memo for more details.
  sync_tree2 : Subsystem
  ten_Gbe_v2 : xps_library/ten_Gbe_v2  Tag=xps:tengbe_v2  flavour=sfp+  slot=0  port_r1=0  port_r2_cx4=0  port_r2_sfpp=0  rx_dist_ram=on  large_frames=on  show_param=on  pre_emph_r2=1.07  pre_emph=3  post_emph_r2=0.18  rxeqmix_r2=7  swing_r2=940  swing=800  fab_en=on  fab_mac=hex2dec('123456780000')  fab_ip=192*(2^24) + 168*(2^16) + 5*(2^8) + 20*(2^0)  fab_udp=10000  fab_gate=1  cpu_rx_en=off  cpu_tx_en=on  ttl=hex2dec('FF')  promisc_mode=off  debug_ctr_width=16  txctr=off  txerrctr=off  txerrctr_len=100  txofctr=off  txfullctr=off  txvldctr=off  txsnaplen=0 - no snap  rxctr=off  rxerrctr=off  rxerrctr_len=100  rxofctr=off  rxbadctr=off  rxvldctr=off  rxeofctr=off  rxsnaplen=0 - no snap
  timestamp : Subsystem  Tag=xps:sw_reg  AncestorBlock=xps_library/software_register  mask(swreg){io_dir=From Processor, io_delay=0, sample_period=1, names=reg, bitwidths=32, bin_pts=0, arith_types=0, sim_port=off, show_format=on}
      mask prompts: io_dir "I/O direction"; io_delay "I/O delay"; sample_period "Sample period"; names "Bitfield names [msb...lsb]"; bitwidths "Bitfield widths"; bin_pts "Bitfield binary pts"; arith_types "Bitfield types, ufix=0, fix=1, bool=2"; sim_port "Provide sim input/output?"; show_format "Print format string?"
      mask help: A 32-bit software-accessible register. Can be divided into bitfields of varying widths and types using the fields in the block mask.
      mask init:
      | try
      |     swreg_init(gcb)
      | catch ex
      |     disp(sprintf('%s: %s', gcb, ex.message))
      |     errordlg(ex.message)
      | end
      settings: AttributesFormatString=1input:uf32.0 = 32 bits
      mask TypeOptions io_dir: To Processor | From Processor
      mask Callback io_dir:
      | mask_enables = get_param(gcb, 'MaskEnables');
      | mask_names = get_param(gcb, 'MaskNames');
      | if strcmp(get_param(gcb, 'io_dir'), 'To Processor'),
      |     mask_enables{ismember(mask_names, 'sample_period')} = 'off';
      | else
      |     mask_enables{ismember(mask_names, 'sample_period')} = 'on';
      | end
      | set_param(gcb, 'MaskEnables', mask_enables);
  ucf : xps_library/ucf  Tag=xps:ucf  ucf_file=/home/Workspace/seba/frb_actual/one_gbe_constrain.ucf
  wires:
  Black Box6/6 -> Terminator1/1
  bus_create/1(bus_out) -> pipeline276/1
  Band-Limited White Noise/1 -> asiaa_adc5g0/1(sim_a)
  Constant13/1 -> asiaa_adc5g0/3(sim_sync)
  sync_gen/1(sync_out) -> [sync_out]
  pipeline276/1 -> adcsnap0/1(din), adc_clip0/2(din)
  Band-Limited White Noise2/1 -> asiaa_adc5g0/2(sim_c)
  asiaa_adc5g0/17(sync_out) -> Terminator/1
  asiaa_adc5g0/1(a0) -> conv_bus4/2(i0)
  asiaa_adc5g0/2(a1) -> conv_bus4/3(i1)
  asiaa_adc5g0/3(a2) -> conv_bus4/4(i2)
  asiaa_adc5g0/4(a3) -> conv_bus4/5(i3)
  asiaa_adc5g0/5(a4) -> conv_bus4/6(i4)
  asiaa_adc5g0/6(a5) -> conv_bus4/7(i5)
  asiaa_adc5g0/7(a6) -> conv_bus4/8(i6)
  asiaa_adc5g0/8(a7) -> conv_bus4/9(i7)
  [cnt_rst] -> acc_cntrl0/3(rst)
  [acc_len] -> acc_cntrl0/1(acc_len)
  pipeline73/1(q) -> simple_bram_vacc_0_0/2(din)
  pre_bram_delay0/2(Out1) -> Reinterpret31/1
  pre_bram_delay0/6(valid_out) -> Counter1/2, antenna_0/3(we)
  pre_bram_delay0/1(sync_out) -> Counter1/1
  pipeline58/1(q) -> simple_bram_vacc_0_0/1(new_acc)
  pipeline60/1(q) -> simple_bram_vacc_0_1/2(din)
  pre_bram_delay0/3(Out2) -> Reinterpret24/1
  pipeline63/1(q) -> simple_bram_vacc_0_1/1(new_acc)
  pipeline64/1(q) -> simple_bram_vacc_0_2/2(din)
  pre_bram_delay0/4(Out3) -> Reinterpret25/1
  pipeline67/1(q) -> simple_bram_vacc_0_2/1(new_acc)
  pipeline68/1(q) -> simple_bram_vacc_0_3/2(din)
  pre_bram_delay0/5(Out4) -> Reinterpret26/1
  pipeline71/1(q) -> simple_bram_vacc_0_3/1(new_acc)
  Delay32/1 -> pipeline73/1(d)
  Delay34/1 -> pipeline60/1(d)
  Delay35/1 -> pipeline64/1(d)
  Delay36/1 -> pipeline68/1(d)
  acc_cntrl0/1(new_acc) -> pipeline71/1(d), pipeline67/1(d), pipeline63/1(d), pipeline58/1(d), pipeline59/1(d)
  post_fft_delay0/1(sync_out) -> antenna_power0/1(sync_in), [sync_out0]
  post_fft_delay0/2(Out1) -> antenna_power0/2(din0), [fft0_0]
  post_fft_delay0/3(Out2) -> antenna_power0/3(din1), [fft0_1]
  post_fft_delay0/4(Out3) -> antenna_power0/4(din2), [fft0_2]
  post_fft_delay0/5(Out4) -> antenna_power0/5(din3), [fft0_3]
  antenna_power0/2(dout0) -> power_convert0/1(In1)
  antenna_power0/3(dout1) -> power_convert0/2(In2)
  antenna_power0/4(dout2) -> power_convert0/3(In3)
  antenna_power0/5(dout3) -> power_convert0/4(In4)
  antenna_power0/1(sync_out) -> pipeline127/1(d)
  [sync_out] -> delay_wideband_prog0/1(sync)
  [snap_trig] -> adcsnap0/2(we), adcsnap0/3(trig)
  [adc0_delay] -> delay_wideband_prog0/2(delay)
  Constant8/1 -> delay_wideband_prog0/3(ld_delay)
  delay_wideband_prog0/9(data_out7) -> pre_pfb_delay1/9(In1)
  delay_wideband_prog0/7(data_out5) -> pre_pfb_delay1/7(In8)
  delay_wideband_prog0/2(data_out0) -> pre_pfb_delay1/2(In3)
  delay_wideband_prog0/3(data_out1) -> pre_pfb_delay1/3(In4)
  delay_wideband_prog0/5(data_out3) -> pre_pfb_delay1/5(In6)
  delay_wideband_prog0/8(data_out6) -> pre_pfb_delay1/8(In9)
  delay_wideband_prog0/4(data_out2) -> pre_pfb_delay1/4(In5)
  delay_wideband_prog0/6(data_out4) -> pre_pfb_delay1/6(In7)
  delay_wideband_prog0/1(sync_out) -> pre_pfb_delay1/1(sync_in)
  conv_bus4/1(q0) -> delay_wideband_prog0/4(data_in0)
  conv_bus4/2(q1) -> delay_wideband_prog0/5(data_in1)
  conv_bus4/3(q2) -> delay_wideband_prog0/6(data_in2)
  conv_bus4/4(q3) -> delay_wideband_prog0/7(data_in3)
  conv_bus4/5(q4) -> delay_wideband_prog0/8(data_in4)
  conv_bus4/6(q5) -> delay_wideband_prog0/9(data_in5)
  conv_bus4/7(q6) -> delay_wideband_prog0/10(data_in6)
  conv_bus4/8(q7) -> delay_wideband_prog0/11(data_in7)
  pre_pfb_delay1/2(Out3) -> bus_create/1(in1), Black Box6/2
  pre_pfb_delay1/3(Out4) -> bus_create/2(in2), Black Box6/3
  pre_pfb_delay1/4(Out5) -> Black Box6/4, bus_create/3(in3)
  pre_pfb_delay1/5(Out6) -> Black Box6/5, bus_create/4(in4)
  pre_pfb_delay1/6(Out7) -> bus_create/5(in5), Black Box6/6
  pre_pfb_delay1/7(Out8) -> Black Box6/7, bus_create/6(in6)
  pre_pfb_delay1/8(Out9) -> bus_create/7(in7), Black Box6/8
  pre_pfb_delay1/9(Out1) -> Black Box6/9, bus_create/8(in8)
  pre_pfb_delay1/1(sync_out) -> Black Box6/1
  Black Box6/5 -> post_fft_delay0/5(In4)
  Black Box6/3 -> post_fft_delay0/3(In2)
  Black Box6/4 -> post_fft_delay0/4(In3)
  Black Box6/2 -> post_fft_delay0/2(In1)
  Black Box6/1 -> post_fft_delay0/1(sync_in)
  pipeline127/1(q) -> acc_cntrl0/2(sync)
  power_convert0/1(Out1) -> Delay32/1
  power_convert0/2(Out2) -> Delay34/1
  power_convert0/3(Out3) -> Delay35/1
  power_convert0/4(Out4) -> Delay36/1
  Concat/1 -> antenna_0/2(data_in)
  Counter1/1 -> antenna_0/1(addr)
  simple_bram_vacc_0_0/1(dout) -> pre_bram_delay0/2(In1)
  simple_bram_vacc_0_1/1(dout) -> pre_bram_delay0/3(In2)
  simple_bram_vacc_0_2/1(dout) -> pre_bram_delay0/4(In3)
  simple_bram_vacc_0_3/1(dout) -> pre_bram_delay0/5(In4)
  simple_bram_vacc_0_3/2(valid) -> pre_bram_delay0/6(valid_in)
  pipeline59/1(q) -> pre_bram_delay0/1(sync_in)
  control/1(cnt_rst) -> [cnt_rst]
  control/2(snap_trig) -> [snap_trig]
  control/3(adc0_delay) -> [adc0_delay]
  control/4(adc1_delay) -> [adc1_delay]
  control/5(adc2_delay) -> [adc2_delay]
  control/6(adc3_delay) -> [adc3_delay]
  control/7(gbe_ip) -> [gbe_ip]
  control/8(gbe_port) -> [gbe_port]
  control/9(tge_ip) -> [tge_ip]
  control/10(tge_port) -> [tge_port]
  control/11(adc_gain) -> [adc_gain]
  control/12(rst_detection) -> [rst_detection]
  [adc_gain] -> conv_bus4/1(gain)
  conv_bus4/9(reduced) -> [adc0]
  beam_post_complex_add/5(Out4) -> concat_order/4(ch3), beam_power/5(din3)
  beam_post_complex_add/4(Out3) -> beam_power/4(din2), concat_order/3(ch2)
  beam_post_complex_add/3(Out2) -> concat_order/2(ch1), beam_power/3(din1)
  beam_post_complex_add/2(Out1) -> concat_order/1(ch0), beam_power/2(din0)
  beam_power/1(sync_out) -> post_flag_delay1/1(sync_in)
  [cnt_rst] -> acc_cntrl4/3(rst)
  [acc_len] -> acc_cntrl4/1(acc_len)
  pipeline11/1(q) -> beam_vacc0/2(din)
  pipeline1/1(q) -> beam_vacc0/1(new_acc)
  pipeline3/1(q) -> beam_vacc1/2(din)
  pipeline5/1(q) -> beam_vacc1/1(new_acc)
  pipeline7/1(q) -> beam_vacc2/2(din)
  pipeline8/1(q) -> beam_vacc2/1(new_acc)
  pipeline9/1(q) -> beam_vacc3/2(din)
  pipeline10/1(q) -> beam_vacc3/1(new_acc)
  Delay2/1 -> pipeline11/1(d)
  Delay3/1 -> pipeline3/1(d)
  Delay4/1 -> pipeline7/1(d)
  Delay5/1 -> pipeline9/1(d)
  acc_cntrl4/1(new_acc) -> pipeline10/1(d), pipeline8/1(d), pipeline5/1(d), pipeline1/1(d), pipeline2/1(d)
  beam_power_conv/1(sync_out) -> acc_cntrl4/2(sync)
  beam_power_conv/2(Out1) -> Delay2/1
  beam_power_conv/3(Out2) -> Delay3/1
  beam_power_conv/4(Out3) -> Delay4/1
  beam_power_conv/5(Out4) -> Delay5/1
  Concat4/1 -> beam/2(data_in)
  Counter5/1 -> beam/1(addr)
  beam_vacc0/1(dout) -> beam_post_acc_delay/2(In1)
  beam_vacc1/1(dout) -> beam_post_acc_delay/3(In2)
  beam_vacc2/1(dout) -> beam_post_acc_delay/4(In3)
  beam_vacc3/1(dout) -> beam_post_acc_delay/5(In4)
  beam_vacc3/2(valid) -> beam_post_acc_delay/6(valid_in)
  pipeline2/1(q) -> beam_post_acc_delay/1(sync_in)
  concat_/1(Out1) -> Mux/2
  beam_post_acc_delay/6(valid_out) -> pipeline23/1(d), Counter5/2, beam/3(we)
  Logical/1 -> pipeline12/1(d)
  Register/1 -> Logical1/1
  pipeline12/1(q) -> Logical1/2
  Inverter/1 -> Register/2
  [tge_en] -> Inverter/1
  Constant6/1 -> ten_Gbe_v2/7
  ten_Gbe_v2/12 -> Delay/1
  Delay/1 -> ten_Gbe_v2/8
  ten_Gbe_v2/1 -> Terminator14/1
  ten_Gbe_v2/2 -> Terminator15/1
  ten_Gbe_v2/4 -> Terminator3/1
  ten_Gbe_v2/5 -> Terminator19/1
  ten_Gbe_v2/6 -> Terminator20/1
  ten_Gbe_v2/7 -> Terminator21/1
  ten_Gbe_v2/8 -> Terminator22/1
  ten_Gbe_v2/9 -> Terminator23/1
  ten_Gbe_v2/10 -> Terminator24/1
  ten_Gbe_v2/11 -> Terminator25/1
  ten_Gbe_v2/13 -> Terminator26/1
  ten_Gbe_v2/14 -> Terminator27/1
  [tge_rst] -> ten_Gbe_v2/1
  pipeline19/1(q) -> concat_/1(In1)
  pipeline20/1(q) -> concat_/2(In2)
  pipeline21/1(q) -> concat_/3(In3)
  pipeline22/1(q) -> concat_/4(In4)
  pipeline23/1(q) -> Logical/2
  beam_post_acc_delay/2(Out1) -> pipeline19/1(d), Reinterpret16/1
  beam_post_acc_delay/5(Out4) -> pipeline22/1(d), Reinterpret15/1
  beam_post_acc_delay/4(Out3) -> pipeline21/1(d), Reinterpret14/1
  beam_post_acc_delay/3(Out2) -> pipeline20/1(d), Reinterpret13/1
  beam_post_acc_delay/1(sync_out) -> pipeline18/1(d), Counter5/1
  pipeline18/1(q) -> Mux/1, Register/3, Register/1, Logical/1
  [header] -> Mux/3
  control/13(tge_pkt) -> [tge_pkt]
  control/14(tge_sleep) -> [tge_sleep]
  control/15(tge_en) -> [tge_en]
  Constant/1 -> Concat5/1
  Constant1/1 -> Concat5/2
  AddSub/1 -> Concat5/3
  Concat10/1 -> pipeline106/1(d)
  Concat5/1 -> [header]
  [rst] -> pipeline421/1
  [rst] -> pipeline422/1
  [gbe_data] -> pipeline423/1
  [gbe_valid] -> pipeline424/1
  [gbe_eof] -> pipeline430/1
  Delay91/1 -> pipeline428/1
  one_GbE/1 -> Terminator59/1
  one_GbE/2 -> Terminator60/1
  one_GbE/3 -> Terminator61/1
  one_GbE/4 -> Terminator53/1
  one_GbE/5 -> Terminator54/1
  one_GbE/6 -> Terminator55/1
  one_GbE/7 -> Terminator56/1
  one_GbE/8 -> Terminator57/1
  one_GbE/9 -> Terminator58/1
  one_GbE/10 -> Terminator51/1
  one_GbE/11 -> Terminator52/1
  Concat6/1 -> pipeline406/1(d)
  ring/1(dout) -> pipeline403/1
  ring/2(eof) -> pipeline404/1
  ring/3(val) -> pipeline405/1
  pipeline407/1 -> Concat6/1
  pipeline408/1 -> Concat6/2
  pipeline409/1 -> Concat6/3
  pipeline406/1(q) -> ring/2(data_in)
  [adc0] -> pipeline407/1
  [adc1] -> pipeline408/1
  [adc2] -> pipeline409/1
  [gbe_port] -> Delay92/1
  [gbe_ip] -> Delay91/1
  control1/1(in_reg) -> Slice12/1, Slice11/1, Slice10/1
  Slice10/1 -> Delay6/1
  Slice11/1 -> Delay49/1
  Delay6/1 -> [write]
  Delay49/1 -> [rst]
  Slice12/1 -> Delay11/1
  Delay11/1 -> [allow_detect]
  [detection] -> Delay93/1
  [write] -> Logical24/2
  Logical23/1 -> Logical24/1
  [allow_detect] -> Inverter3/1
  Logical24/1 -> ring/1(write_en)
  Inverter3/1 -> Logical23/1
  pipeline403/1 -> [gbe_data]
  pipeline404/1 -> [gbe_eof]
  pipeline405/1 -> [gbe_valid]
  Delay93/1 -> Logical23/2
  pipeline421/1 -> one_GbE/1
  pipeline422/1 -> one_GbE/2
  pipeline423/1 -> one_GbE/3
  pipeline424/1 -> one_GbE/4
  pipeline428/1 -> one_GbE/5
  pipeline429/1 -> one_GbE/6
  pipeline430/1 -> one_GbE/7
  Delay92/1 -> pipeline429/1
  Constant105/1 -> one_GbE/8
  Logical3/1 -> [detection]
  control/16(rst_tge) -> [tge_rst]
  beam_post_complex_add/1(sync_out) -> beam_power/1(sync_in), Black Box5/1
  concat_order/1(Out1) -> Black Box5/2
  [flag_rfi] -> Black Box5/3
  [flag_num] -> Black Box5/4
  [flag_en] -> Black Box5/5
  Counter6/1 -> Slice8/1, Slice7/1, Slice6/1
  Slice6/1 -> Logical2/2
  Slice7/1 -> Logical2/3
  Subsystem3/1(Out1) -> pre_dedisp_acc_conv/2(din)
  Slice8/1 -> Logical2/1
  Logical2/1 -> pre_dedisp_acc_conv/3(din_valid)
  adder_tree1/1(sync_out) -> pre_dedisp_acc_conv/1(sync_in), Counter6/1
  adder_tree1/2(dout) -> Subsystem3/1(In1)
  Black Box5/2 -> Slice9/1, Slice2/1, Slice5/1, Slice3/1, Slice1/1, Slice4/1, Slice16/1, Slice17/1
  Black Box5/1 -> Convert5/1, Convert46/1
  Convert46/1 -> post_flag_delay/1(sync_in)
  Slice4/1 -> post_flag_delay/2(In1)
  Slice9/1 -> post_flag_delay/3(In2)
  Slice16/1 -> post_flag_delay/4(In3)
  Slice17/1 -> post_flag_delay/5(In4)
  post_flag_delay/2(Out1) -> flag_power/2(din0)
  post_flag_delay/4(Out3) -> flag_power/4(din2)
  post_flag_delay/3(Out2) -> flag_power/3(din1)
  post_flag_delay/1(sync_out) -> flag_power/1(sync_in)
  post_flag_delay/5(Out4) -> flag_power/5(din3)
  flag_power/5(dout3) -> flag_convert/5(In4)
  flag_power/1(sync_out) -> flag_convert/1(sync_in)
  flag_power/4(dout2) -> flag_convert/4(In3)
  flag_power/2(dout0) -> flag_convert/2(In1)
  flag_power/3(dout1) -> flag_convert/3(In2)
  flag_convert/1(sync_out) -> adder_tree1/1(sync)
  flag_convert/3(Out2) -> adder_tree1/3(din2)
  flag_convert/5(Out4) -> adder_tree1/5(din4)
  flag_convert/2(Out1) -> adder_tree1/2(din1)
  flag_convert/4(Out3) -> adder_tree1/4(din3)
  control/17(flag_en) -> [flag_en]
  control/18(flag_num) -> [flag_num]
  control/19(flag_rfi) -> [flag_rfi]
  control/20(acc_len0) -> [acc_len]
  control/21(acc_len1) -> [acc_len0]
  control/22(acc_len2) -> [acc_len1]
  control/23(acc_len3) -> [acc_len2]
  control/24(acc_len4) -> [acc_len3]
  Reinterpret31/1 -> Concat/1
  Reinterpret24/1 -> Concat/2
  Reinterpret25/1 -> Concat/3
  Reinterpret26/1 -> Concat/4
  Reinterpret16/1 -> Concat4/1
  Reinterpret13/1 -> Concat4/2
  Reinterpret14/1 -> Concat4/3
  Reinterpret15/1 -> Concat4/4
  pipeline30/1 -> sync_tree2/1(In1)
  pipeline53/1 -> m0_tree2/1(In1)
  pipeline27/1 -> m0_en1/1(In1)
  pre_dedisp_acc_conv/2(dout) -> pipeline53/1
  pre_dedisp_acc_conv/1(sync_out) -> pipeline30/1
  pre_dedisp_acc_conv/3(dout_valid) -> pipeline27/1
  control/33(rst_dedisp) -> [rst_dedisp]
  control/35(theta1) -> [theta0]
  control/36(theta2) -> [theta1]
  control/37(theta3) -> [theta2]
  control/38(theta4) -> [theta3]
  [acc_len0] -> acc_cntrl5/1(acc_len)
  [sd0] -> acc_cntrl5/2(sync)
  [cnt_rst] -> acc_cntrl5/3(rst)
  Logical27/1 -> enabled_vacc0/1(new_acc), pipeline24/1(d), Register16/3, Register16/1
  pipeline15/1(q) -> enabled_vacc0/2(din)
  [m0e0] -> pipeline16/1(d)
  [m0d0] -> pipeline15/1(d)
  enabled_vacc0/1(dout) -> Convert2/1, pre_dedisp_conv0/1(din)
  enabled_vacc0/2(dout_valid) -> pipeline17/1(d), pre_dedisp_conv0/2(din_valid)
  pre_dedisp_conv0/2(dout_valid) -> pre_dedisp_delay0/2(din_valid)
  pre_dedisp_conv0/1(dout) -> pre_dedisp_delay0/1(In1)
  pre_dedisp_delay0/2(dout_valid) -> dedispersor0/3(din_valid)
  pre_dedisp_delay0/1(Out1) -> dedispersor0/2(din)
  [rst_dedisp] -> dedispersor0/1(rst)
  dedispersor0/1(integ_pow) -> post_dedisp_conv0/1(din)
  dedispersor0/2(integ_valid) -> post_dedisp_conv0/2(din_valid)
  post_dedisp_conv0/1(dout) -> post_dedisp_delay0/1(In1)
  post_dedisp_conv0/2(dout_valid) -> post_dedisp_delay0/2(din_valid)
  post_dedisp_delay0/1(Out1) -> Convert3/1, Relational/1, mov_avg0/2(din)
  [rst_dedisp] -> mov_avg0/1(rst)
  mov_avg0/1(dout) -> add_stat0/2
  add_stat0/1 -> Relational/2, Convert4/1
  [theta0] -> add_stat0/1
  Logical11/1 -> pipeline42/1
  [rst_detection] -> Register2/2
  Register2/1 -> [detection0]
  Convert2/1 -> Reinterpret17/1
  Reinterpret17/1 -> debug_acc/2(data_in)
  pipeline24/1(q) -> Counter7/1
  pipeline17/1(q) -> Counter7/2, debug_acc/3(we)
  Counter7/1 -> debug_acc/1(addr)
  Counter8/1 -> dedisp0/1(addr)
  post_dedisp_delay0/2(dout_valid) -> pipeline75/1(d), Counter8/1, dedisp0/3(we), mov_avg0/3(din_valid)
  Convert3/1 -> Reinterpret19/1
  Reinterpret19/1 -> dedisp0/2(data_in)
  Counter9/1 -> avg0/1(addr)
  mov_avg0/2(dout_valid) -> Counter9/1, avg0/3(we)
  Convert4/1 -> Reinterpret20/1
  Reinterpret20/1 -> avg0/2(data_in)
  Convert5/1 -> beam_rfi_delay/1(sync_in)
  Slice3/1 -> beam_rfi_delay/2(In1)
  Slice5/1 -> beam_rfi_delay/3(In2)
  Slice1/1 -> beam_rfi_delay/4(In3)
  Slice2/1 -> beam_rfi_delay/5(In4)
  beam_rfi_delay/1(sync_out) -> [beam_sync]
  beam_rfi_delay/2(Out1) -> [beam0]
  beam_rfi_delay/3(Out2) -> [beam1]
  beam_rfi_delay/4(Out3) -> [beam2]
  beam_rfi_delay/5(Out4) -> [beam3]
  [tge_rst] -> packetizer/1(rst)
  Mux/1 -> packetizer/2(din)
  [tge_pkt] -> packetizer/3(pkt_len)
  [tge_sleep] -> packetizer/4(sleep_cycle)
  [tge_ip] -> packetizer/5(config_tx_dest_ip)
  Logical1/1 -> packetizer/6(din_valid)
  [tge_port] -> packetizer/7(config_tx_dest_port)
  packetizer/1(tx_data) -> ten_Gbe_v2/2
  packetizer/2(tx_valid) -> ten_Gbe_v2/3
  packetizer/3(tx_dest_ip) -> ten_Gbe_v2/4
  packetizer/4(tx_dest_port) -> ten_Gbe_v2/5
  packetizer/5(tx_eof) -> ten_Gbe_v2/6
  [acc_len1] -> acc_cntrl6/1(acc_len)
  [sd0] -> acc_cntrl6/2(sync)
  [cnt_rst] -> acc_cntrl6/3(rst)
  pipeline33/1(q) -> enabled_vacc1/2(din)
  [m0e1] -> pipeline34/1(d)
  [m0d1] -> pipeline33/1(d)
  enabled_vacc1/1(dout) -> pre_dedisp_conv1/1(din)
  enabled_vacc1/2(dout_valid) -> pre_dedisp_conv1/2(din_valid)
  pre_dedisp_conv1/2(dout_valid) -> pre_dedisp_delay1/2(din_valid)
  pre_dedisp_conv1/1(dout) -> pre_dedisp_delay1/1(In1)
  pre_dedisp_delay1/2(dout_valid) -> dedispersor1/3(din_valid)
  pre_dedisp_delay1/1(Out1) -> dedispersor1/2(din)
  [rst_dedisp] -> dedispersor1/1(rst)
  dedispersor1/1(integ_pow) -> post_dedisp_conv1/1(din)
  dedispersor1/2(integ_valid) -> post_dedisp_conv1/2(din_valid)
  post_dedisp_conv1/1(dout) -> post_dedisp_delay1/1(In1)
  post_dedisp_conv1/2(dout_valid) -> post_dedisp_delay1/2(din_valid)
  post_dedisp_delay1/1(Out1) -> Convert7/1, Relational1/1, mov_avg1/2(din)
  [rst_dedisp] -> mov_avg1/1(rst)
  mov_avg1/1(dout) -> add_stat1/2
  add_stat1/1 -> Relational1/2, Convert8/1
  [theta1] -> add_stat1/1
  [rst_detection] -> Register3/2
  Register3/1 -> [detection1]
  Counter13/1 -> dedisp1/1(addr)
  post_dedisp_delay1/2(dout_valid) -> Counter13/1, pipeline79/1(d), dedisp1/3(we), mov_avg1/3(din_valid)
  Convert7/1 -> Reinterpret35/1
  Reinterpret35/1 -> dedisp1/2(data_in)
  Counter14/1 -> avg1/1(addr)
  mov_avg1/2(dout_valid) -> Counter14/1, avg1/3(we)
  Convert8/1 -> Reinterpret36/1
  Reinterpret36/1 -> avg1/2(data_in)
  [acc_len2] -> acc_cntrl7/1(acc_len)
  [sd0] -> acc_cntrl7/2(sync)
  [cnt_rst] -> acc_cntrl7/3(rst)
  pipeline35/1(q) -> enabled_vacc2/2(din)
  [m0e2] -> pipeline36/1(d)
  [m0d2] -> pipeline35/1(d)
  enabled_vacc2/1(dout) -> pre_dedisp_conv2/1(din)
  enabled_vacc2/2(dout_valid) -> pre_dedisp_conv2/2(din_valid)
  pre_dedisp_conv2/2(dout_valid) -> pre_dedisp_delay2/2(din_valid)
  pre_dedisp_conv2/1(dout) -> pre_dedisp_delay2/1(In1)
  pre_dedisp_delay2/2(dout_valid) -> dedispersor2/3(din_valid)
  pre_dedisp_delay2/1(Out1) -> dedispersor2/2(din)
  [rst_dedisp] -> dedispersor2/1(rst)
  dedispersor2/1(integ_pow) -> post_dedisp_conv2/1(din)
  dedispersor2/2(integ_valid) -> post_dedisp_conv2/2(din_valid)
  post_dedisp_conv2/1(dout) -> post_dedisp_delay2/1(In1)
  post_dedisp_conv2/2(dout_valid) -> post_dedisp_delay2/2(din_valid)
  post_dedisp_delay2/1(Out1) -> Convert6/1, Relational2/1, mov_avg2/2(din)
  [rst_dedisp] -> mov_avg2/1(rst)
  mov_avg2/1(dout) -> add_stat2/2
  add_stat2/1 -> Relational2/2, Convert9/1
  [theta2] -> add_stat2/1
  [rst_detection] -> Register4/2
  Register4/1 -> [detection2]
  Counter12/1 -> dedisp2/1(addr)
  post_dedisp_delay2/2(dout_valid) -> Counter12/1, pipeline80/1(d), dedisp2/3(we), mov_avg2/3(din_valid)
  Convert6/1 -> Reinterpret37/1
  Reinterpret37/1 -> dedisp2/2(data_in)
  Counter15/1 -> avg2/1(addr)
  mov_avg2/2(dout_valid) -> Counter15/1, avg2/3(we)
  Convert9/1 -> Reinterpret38/1
  Reinterpret38/1 -> avg2/2(data_in)
  [acc_len3] -> acc_cntrl8/1(acc_len)
  [sd0] -> acc_cntrl8/2(sync)
  [cnt_rst] -> acc_cntrl8/3(rst)
  pipeline37/1(q) -> enabled_vacc3/2(din)
  [m0e3] -> pipeline38/1(d)
  [m0d3] -> pipeline37/1(d)
  enabled_vacc3/1(dout) -> pre_dedisp_conv3/1(din)
  enabled_vacc3/2(dout_valid) -> pre_dedisp_conv3/2(din_valid)
  pre_dedisp_conv3/2(dout_valid) -> pre_dedisp_delay3/2(din_valid)
  pre_dedisp_conv3/1(dout) -> pre_dedisp_delay3/1(In1)
  pre_dedisp_delay3/2(dout_valid) -> dedispersor3/3(din_valid)
  pre_dedisp_delay3/1(Out1) -> dedispersor3/2(din)
  [rst_dedisp] -> dedispersor3/1(rst)
  dedispersor3/1(integ_pow) -> post_dedisp_conv3/1(din)
  dedispersor3/2(integ_valid) -> post_dedisp_conv3/2(din_valid)
  post_dedisp_conv3/1(dout) -> post_dedisp_delay3/1(In1)
  post_dedisp_conv3/2(dout_valid) -> post_dedisp_delay3/2(din_valid)
  post_dedisp_delay3/1(Out1) -> Convert10/1, Relational3/1, mov_avg3/2(din)
  [rst_dedisp] -> mov_avg3/1(rst)
  mov_avg3/1(dout) -> add_stat3/2
  add_stat3/1 -> Relational3/2, Convert11/1
  [theta3] -> add_stat3/1
  [rst_detection] -> Register5/2
  Register5/1 -> [detection3]
  Counter16/1 -> dedisp3/1(addr)
  post_dedisp_delay3/2(dout_valid) -> Counter16/1, pipeline83/1(d), dedisp3/3(we), mov_avg3/3(din_valid)
  Convert10/1 -> Reinterpret40/1
  Reinterpret40/1 -> dedisp3/2(data_in)
  Counter17/1 -> avg3/1(addr)
  mov_avg3/2(dout_valid) -> Counter17/1, avg3/3(we)
  Convert11/1 -> Reinterpret41/1
  Reinterpret41/1 -> avg3/2(data_in)
  [detection0] -> Logical3/1
  [detection1] -> Logical3/2
  [detection2] -> Logical3/3
  [detection3] -> Logical3/4
  pipeline39/1 -> Register5/3, Register5/1
  pipeline40/1 -> Register4/3, Register4/1
  pipeline41/1 -> Register3/3, Register3/1
  pipeline42/1 -> Register2/3, Register2/1
  [acc_len4] -> acc_cntrl9/1(acc_len)
  [sd0] -> acc_cntrl9/2(sync)
  [cnt_rst] -> acc_cntrl9/3(rst)
  pipeline43/1(q) -> enabled_vacc4/2(din)
  [m0e4] -> pipeline45/1(d)
  [m0d4] -> pipeline43/1(d)
  enabled_vacc4/1(dout) -> pre_dedisp_conv4/1(din)
  enabled_vacc4/2(dout_valid) -> pre_dedisp_conv4/2(din_valid)
  pre_dedisp_conv4/2(dout_valid) -> pre_dedisp_delay4/2(din_valid)
  pre_dedisp_conv4/1(dout) -> pre_dedisp_delay4/1(In1)
  pre_dedisp_delay4/2(dout_valid) -> dedispersor4/3(din_valid)
  pre_dedisp_delay4/1(Out1) -> dedispersor4/2(din)
  [rst_dedisp] -> dedispersor4/1(rst)
  dedispersor4/1(integ_pow) -> post_dedisp_conv4/1(din)
  dedispersor4/2(integ_valid) -> post_dedisp_conv4/2(din_valid)
  post_dedisp_conv4/1(dout) -> post_dedisp_delay4/1(In1)
  post_dedisp_conv4/2(dout_valid) -> post_dedisp_delay4/2(din_valid)
  post_dedisp_delay4/1(Out1) -> Convert12/1, Relational4/1, mov_avg4/2(din)
  [rst_dedisp] -> mov_avg4/1(rst)
  mov_avg4/1(dout) -> add_stat4/2
  add_stat4/1 -> Relational4/2, Convert13/1
  [theta4] -> add_stat4/1
  [rst_detection] -> Register6/2
  Register6/1 -> [detection4]
  Counter18/1 -> dedisp4/1(addr)
  post_dedisp_delay4/2(dout_valid) -> Counter18/1, pipeline84/1(d), dedisp4/3(we), mov_avg4/3(din_valid)
  Convert12/1 -> Reinterpret43/1
  Reinterpret43/1 -> dedisp4/2(data_in)
  Counter19/1 -> avg4/1(addr)
  mov_avg4/2(dout_valid) -> Counter19/1, avg4/3(we)
  Convert13/1 -> Reinterpret44/1
  Reinterpret44/1 -> avg4/2(data_in)
  pipeline46/1 -> Register6/3, Register6/1
  [detection4] -> Logical3/5
  control/25(acc_len5) -> [acc_len4]
  control/39(theta5) -> [theta4]
  control/47(rfi_acc_len) -> [rfi_acc_len]
  control/49(rfi_en) -> [rfi_en]
  control/50(rfi_hold) -> [rfi_hold]
  control/48(rfi_thresh) -> [rfi_thresh]
  Relational/1 -> Logical11/2
  [rfi_detected] -> Inverter2/1
  Logical12/1 -> pipeline41/1
  Relational1/1 -> Logical12/2
  [rfi_detected] -> Inverter4/1
  Logical13/1 -> pipeline40/1
  Relational2/1 -> Logical13/2
  [rfi_detected] -> Inverter5/1
  Logical14/1 -> pipeline39/1
  Relational3/1 -> Logical14/2
  [rfi_detected] -> Inverter6/1
  Logical15/1 -> pipeline46/1
  Relational4/1 -> Logical15/2
  [rfi_detected] -> Inverter7/1
  control/34(en_dedisp) -> [en_dedisp]
  Logical16/1 -> enabled_vacc1/1(new_acc), Register12/3, Register12/1
  acc_cntrl6/1(new_acc) -> Logical16/2
  [en_dedisp] -> Logical16/1
  Register12/1 -> Logical25/1
  [rst_dedisp] -> Register12/2
  Logical17/1 -> Register13/3, Register13/1, enabled_vacc2/1(new_acc)
  acc_cntrl7/1(new_acc) -> Logical17/2
  [en_dedisp] -> Logical17/1
  Register13/1 -> Logical22/1
  [rst_dedisp] -> Register13/2
  Logical18/1 -> enabled_vacc3/1(new_acc), Register14/3, Register14/1
  acc_cntrl8/1(new_acc) -> Logical18/2
  [en_dedisp] -> Logical18/1
  Register14/1 -> Logical20/1
  [rst_dedisp] -> Register14/2
  Logical19/1 -> Register15/3, Register15/1, enabled_vacc4/1(new_acc)
  acc_cntrl9/1(new_acc) -> Logical19/2
  [en_dedisp] -> Logical19/1
  Register15/1 -> Logical21/1
  [rst_dedisp] -> Register15/2
  Logical20/1 -> enabled_vacc3/3(din_valid)
  pipeline38/1(q) -> Logical20/2
  Logical21/1 -> enabled_vacc4/3(din_valid)
  pipeline45/1(q) -> Logical21/2
  Logical22/1 -> enabled_vacc2/3(din_valid)
  pipeline36/1(q) -> Logical22/2
  Logical25/1 -> enabled_vacc1/3(din_valid)
  pipeline34/1(q) -> Logical25/2
  Logical26/1 -> enabled_vacc0/3(din_valid)
  pipeline16/1(q) -> Logical26/2
  acc_cntrl5/1(new_acc) -> Logical27/2
  [en_dedisp] -> Logical27/1
  [rst_dedisp] -> Register16/2
  Register16/1 -> Logical26/1
  [acc_len5] -> acc_cntrl10/1(acc_len)
  [sd0] -> acc_cntrl10/2(sync)
  [cnt_rst] -> acc_cntrl10/3(rst)
  pipeline14/1(q) -> enabled_vacc5/2(din)
  [m0e5] -> pipeline26/1(d)
  [m0d5] -> pipeline14/1(d)
  enabled_vacc5/1(dout) -> pre_dedisp_conv5/1(din)
  enabled_vacc5/2(dout_valid) -> pre_dedisp_conv5/2(din_valid)
  pre_dedisp_conv5/2(dout_valid) -> pre_dedisp_delay5/2(din_valid)
  pre_dedisp_conv5/1(dout) -> pre_dedisp_delay5/1(In1)
  pre_dedisp_delay5/2(dout_valid) -> dedispersor5/3(din_valid)
  pre_dedisp_delay5/1(Out1) -> dedispersor5/2(din)
  [rst_dedisp] -> dedispersor5/1(rst)
  dedispersor5/1(integ_pow) -> post_dedisp_conv5/1(din)
  dedispersor5/2(integ_valid) -> post_dedisp_conv5/2(din_valid)
  post_dedisp_conv5/1(dout) -> post_dedisp_delay5/1(In1)
  post_dedisp_conv5/2(dout_valid) -> post_dedisp_delay5/2(din_valid)
  post_dedisp_delay5/1(Out1) -> Convert1/1, Relational10/1, mov_avg5/2(din)
  [rst_dedisp] -> mov_avg5/1(rst)
  mov_avg5/1(dout) -> add_stat5/2
  add_stat5/1 -> Relational10/2, Convert22/1
  [theta5] -> add_stat5/1
  [rst_detection] -> Register18/2
  Register18/1 -> [detection5]
  Counter21/1 -> dedisp5/1(addr)
  post_dedisp_delay5/2(dout_valid) -> Counter21/1, dedisp5/3(we), pipeline87/1(d), mov_avg5/3(din_valid)
  Convert1/1 -> Reinterpret18/1
  Reinterpret18/1 -> dedisp5/2(data_in)
  Counter22/1 -> avg5/1(addr)
  mov_avg5/2(dout_valid) -> Counter22/1, avg5/3(we)
  Convert22/1 -> Reinterpret33/1
  Reinterpret33/1 -> avg5/2(data_in)
  pipeline28/1 -> Register18/3, Register18/1
  Logical28/1 -> pipeline28/1
  Relational10/1 -> Logical28/2
  [rfi_detected] -> Inverter8/1
  Logical29/1 -> Register17/3, Register17/1, enabled_vacc5/1(new_acc)
  acc_cntrl10/1(new_acc) -> Logical29/2
  [en_dedisp] -> Logical29/1
  Register17/1 -> Logical30/1
  [rst_dedisp] -> Register17/2
  Logical30/1 -> enabled_vacc5/3(din_valid)
  pipeline26/1(q) -> Logical30/2
  [detection5] -> Logical3/6
  control/26(acc_len6) -> [acc_len5]
  control/40(theta6) -> [theta5]
  pipeline298/1 -> bus_expand/1(bus_in)
  Constant4/1 -> snapshot/2(we), snapshot/3(trig)
  bus_expand/1(msb_out8) -> Convert25/1
  bus_expand/2(out7) -> Convert26/1
  bus_expand/3(out6) -> Convert27/1
  bus_expand/4(out5) -> Convert28/1
  bus_expand/5(out4) -> Convert29/1
  bus_expand/6(out3) -> Convert30/1
  bus_expand/7(out2) -> Convert23/1
  bus_expand/8(lsb_out1) -> Convert24/1
  Convert24/1 -> bus_create4/8(in8)
  Convert23/1 -> bus_create4/7(in7)
  Convert30/1 -> bus_create4/6(in6)
  Convert29/1 -> bus_create4/5(in5)
  Convert28/1 -> bus_create4/4(in4)
  Convert27/1 -> bus_create4/3(in3)
  Convert26/1 -> bus_create4/2(in2)
  Convert25/1 -> bus_create4/1(in1)
  bus_create4/1(bus_out) -> pipeline29/1
  [adc0] -> pipeline298/1
  pipeline29/1 -> snapshot/1(din)
  [acc_len6] -> acc_cntrl11/1(acc_len)
  [sd0] -> acc_cntrl11/2(sync)
  [cnt_rst] -> acc_cntrl11/3(rst)
  pipeline31/1(q) -> enabled_vacc6/2(din)
  [m0e6] -> pipeline32/1(d)
  [m0d6] -> pipeline31/1(d)
  enabled_vacc6/1(dout) -> pre_dedisp_conv6/1(din)
  enabled_vacc6/2(dout_valid) -> pre_dedisp_conv6/2(din_valid)
  pre_dedisp_conv6/2(dout_valid) -> pre_dedisp_delay6/2(din_valid)
  pre_dedisp_conv6/1(dout) -> pre_dedisp_delay6/1(In1)
  pre_dedisp_delay6/2(dout_valid) -> dedispersor6/3(din_valid)
  pre_dedisp_delay6/1(Out1) -> dedispersor6/2(din)
  [rst_dedisp] -> dedispersor6/1(rst)
  dedispersor6/1(integ_pow) -> post_dedisp_conv6/1(din)
  dedispersor6/2(integ_valid) -> post_dedisp_conv6/2(din_valid)
  post_dedisp_conv6/1(dout) -> post_dedisp_delay6/1(In1)
  post_dedisp_conv6/2(dout_valid) -> post_dedisp_delay6/2(din_valid)
  post_dedisp_delay6/1(Out1) -> Convert31/1, Relational11/1, mov_avg6/2(din)
  [rst_dedisp] -> mov_avg6/1(rst)
  mov_avg6/1(dout) -> add_stat6/2
  add_stat6/1 -> Relational11/2, Convert32/1
  [theta6] -> add_stat6/1
  [rst_detection] -> Register20/2
  Register20/1 -> [detection6]
  Counter23/1 -> dedisp6/1(addr)
  post_dedisp_delay6/2(dout_valid) -> Counter23/1, dedisp6/3(we), pipeline88/1(d), mov_avg6/3(din_valid)
  Convert31/1 -> Reinterpret34/1
  Reinterpret34/1 -> dedisp6/2(data_in)
  Counter24/1 -> avg6/1(addr)
  mov_avg6/2(dout_valid) -> Counter24/1, avg6/3(we)
  Convert32/1 -> Reinterpret39/1
  Reinterpret39/1 -> avg6/2(data_in)
  pipeline47/1 -> Register20/3, Register20/1
  Logical31/1 -> pipeline47/1
  Relational11/1 -> Logical31/2
  [rfi_detected] -> Inverter9/1
  Logical32/1 -> Register19/3, Register19/1, enabled_vacc6/1(new_acc)
  acc_cntrl11/1(new_acc) -> Logical32/2
  [en_dedisp] -> Logical32/1
  Register19/1 -> Logical33/1
  [rst_dedisp] -> Register19/2
  Logical33/1 -> enabled_vacc6/3(din_valid)
  pipeline32/1(q) -> Logical33/2
  [detection6] -> Logical3/7
  control/27(acc_len7) -> [acc_len6]
  control/41(theta7) -> [theta6]
  beam_power/3(dout1) -> post_flag_delay1/3(In2)
  beam_power/4(dout2) -> post_flag_delay1/4(In3)
  beam_power/2(dout0) -> post_flag_delay1/2(In1)
  beam_power/5(dout3) -> post_flag_delay1/5(In4)
  post_flag_delay1/4(Out3) -> beam_power_conv/4(In3)
  post_flag_delay1/2(Out1) -> beam_power_conv/2(In1)
  post_flag_delay1/3(Out2) -> beam_power_conv/3(In2)
  post_flag_delay1/1(sync_out) -> beam_power_conv/1(sync_in)
  post_flag_delay1/5(Out4) -> beam_power_conv/5(In4)
  [acc_len7] -> acc_cntrl12/1(acc_len)
  [sd0] -> acc_cntrl12/2(sync)
  [cnt_rst] -> acc_cntrl12/3(rst)
  pipeline48/1(q) -> enabled_vacc7/2(din)
  [m0e7] -> pipeline51/1(d)
  [m0d7] -> pipeline48/1(d)
  enabled_vacc7/1(dout) -> pre_dedisp_conv7/1(din)
  enabled_vacc7/2(dout_valid) -> pre_dedisp_conv7/2(din_valid)
  pre_dedisp_conv7/2(dout_valid) -> pre_dedisp_delay7/2(din_valid)
  pre_dedisp_conv7/1(dout) -> pre_dedisp_delay7/1(In1)
  pre_dedisp_delay7/2(dout_valid) -> dedispersor7/3(din_valid)
  pre_dedisp_delay7/1(Out1) -> dedispersor7/2(din)
  [rst_dedisp] -> dedispersor7/1(rst)
  dedispersor7/1(integ_pow) -> post_dedisp_conv7/1(din)
  dedispersor7/2(integ_valid) -> post_dedisp_conv7/2(din_valid)
  post_dedisp_conv7/1(dout) -> post_dedisp_delay7/1(In1)
  post_dedisp_conv7/2(dout_valid) -> post_dedisp_delay7/2(din_valid)
  post_dedisp_delay7/1(Out1) -> Convert33/1, Relational12/1, mov_avg7/2(din)
  [rst_dedisp] -> mov_avg7/1(rst)
  mov_avg7/1(dout) -> add_stat7/2
  add_stat7/1 -> Relational12/2, Convert34/1
  [theta7] -> add_stat7/1
  [rst_detection] -> Register22/2
  Register22/1 -> [detection7]
  Counter25/1 -> dedisp7/1(addr)
  post_dedisp_delay7/2(dout_valid) -> Counter25/1, dedisp7/3(we), pipeline90/1(d), mov_avg7/3(din_valid)
  Convert33/1 -> Reinterpret42/1
  Reinterpret42/1 -> dedisp7/2(data_in)
  Counter26/1 -> avg7/1(addr)
  mov_avg7/2(dout_valid) -> Counter26/1, avg7/3(we)
  Convert34/1 -> Reinterpret49/1
  Reinterpret49/1 -> avg7/2(data_in)
  pipeline54/1 -> Register22/3, Register22/1
  Logical34/1 -> pipeline54/1
  Relational12/1 -> Logical34/2
  [rfi_detected] -> Inverter10/1
  Logical35/1 -> Register21/3, Register21/1, enabled_vacc7/1(new_acc)
  acc_cntrl12/1(new_acc) -> Logical35/2
  [en_dedisp] -> Logical35/1
  Register21/1 -> Logical36/1
  [rst_dedisp] -> Register21/2
  Logical36/1 -> enabled_vacc7/3(din_valid)
  pipeline51/1(q) -> Logical36/2
  control/42(theta8) -> [theta7]
  control/28(acc_len8) -> [acc_len7]
  [detection7] -> Logical3/8
  [acc_len8] -> acc_cntrl13/1(acc_len)
  [sd0] -> acc_cntrl13/2(sync)
  [cnt_rst] -> acc_cntrl13/3(rst)
  pipeline56/1(q) -> enabled_vacc8/2(din)
  [m0e8] -> pipeline57/1(d)
  [m0d8] -> pipeline56/1(d)
  enabled_vacc8/1(dout) -> pre_dedisp_conv8/1(din)
  enabled_vacc8/2(dout_valid) -> pre_dedisp_conv8/2(din_valid)
  pre_dedisp_conv8/2(dout_valid) -> pre_dedisp_delay8/2(din_valid)
  pre_dedisp_conv8/1(dout) -> pre_dedisp_delay8/1(In1)
  pre_dedisp_delay8/2(dout_valid) -> dedispersor8/3(din_valid)
  pre_dedisp_delay8/1(Out1) -> dedispersor8/2(din)
  [rst_dedisp] -> dedispersor8/1(rst)
  dedispersor8/1(integ_pow) -> post_dedisp_conv8/1(din)
  dedispersor8/2(integ_valid) -> post_dedisp_conv8/2(din_valid)
  post_dedisp_conv8/1(dout) -> post_dedisp_delay8/1(In1)
  post_dedisp_conv8/2(dout_valid) -> post_dedisp_delay8/2(din_valid)
  post_dedisp_delay8/1(Out1) -> Convert35/1, Relational13/1, mov_avg8/2(din)
  [rst_dedisp] -> mov_avg8/1(rst)
  mov_avg8/1(dout) -> add_stat8/2
  add_stat8/1 -> Relational13/2, Convert36/1
  [theta8] -> add_stat8/1
  [rst_detection] -> Register24/2
  Register24/1 -> [detection8]
  Counter27/1 -> dedisp8/1(addr)
  post_dedisp_delay8/2(dout_valid) -> Counter27/1, dedisp8/3(we), pipeline92/1(d), mov_avg8/3(din_valid)
  Convert35/1 -> Reinterpret50/1
  Reinterpret50/1 -> dedisp8/2(data_in)
  Counter28/1 -> avg8/1(addr)
  mov_avg8/2(dout_valid) -> Counter28/1, avg8/3(we)
  Convert36/1 -> Reinterpret51/1
  Reinterpret51/1 -> avg8/2(data_in)
  pipeline61/1 -> Register24/3, Register24/1
  Logical37/1 -> pipeline61/1
  Relational13/1 -> Logical37/2
  [rfi_detected] -> Inverter11/1
  Logical38/1 -> Register23/3, Register23/1, enabled_vacc8/1(new_acc)
  acc_cntrl13/1(new_acc) -> Logical38/2
  [en_dedisp] -> Logical38/1
  Register23/1 -> Logical39/1
  [rst_dedisp] -> Register23/2
  Logical39/1 -> enabled_vacc8/3(din_valid)
  pipeline57/1(q) -> Logical39/2
  [detection8] -> Logical3/9
  control/29(acc_len9) -> [acc_len8]
  control/43(theta9) -> [theta8]
  [acc_len9] -> acc_cntrl14/1(acc_len)
  [sd0] -> acc_cntrl14/2(sync)
  [cnt_rst] -> acc_cntrl14/3(rst)
  pipeline62/1(q) -> enabled_vacc9/2(din)
  [m0e9] -> pipeline65/1(d)
  [m0d9] -> pipeline62/1(d)
  enabled_vacc9/1(dout) -> pre_dedisp_conv9/1(din)
  enabled_vacc9/2(dout_valid) -> pre_dedisp_conv9/2(din_valid)
  pre_dedisp_conv9/2(dout_valid) -> pre_dedisp_delay9/2(din_valid)
  pre_dedisp_conv9/1(dout) -> pre_dedisp_delay9/1(In1)
  pre_dedisp_delay9/2(dout_valid) -> dedispersor9/3(din_valid)
  pre_dedisp_delay9/1(Out1) -> dedispersor9/2(din)
  [rst_dedisp] -> dedispersor9/1(rst)
  dedispersor9/1(integ_pow) -> post_dedisp_conv9/1(din)
  dedispersor9/2(integ_valid) -> post_dedisp_conv9/2(din_valid)
  post_dedisp_conv9/1(dout) -> post_dedisp_delay9/1(In1)
  post_dedisp_conv9/2(dout_valid) -> post_dedisp_delay9/2(din_valid)
  post_dedisp_delay9/1(Out1) -> Convert37/1, Relational14/1, mov_avg9/2(din)
  [rst_dedisp] -> mov_avg9/1(rst)
  mov_avg9/1(dout) -> add_stat9/2
  add_stat9/1 -> Relational14/2, Convert38/1
  [theta9] -> add_stat9/1
  [rst_detection] -> Register26/2
  Register26/1 -> [detection9]
  Counter29/1 -> dedisp9/1(addr)
  post_dedisp_delay9/2(dout_valid) -> mov_avg9/3(din_valid), Counter29/1, pipeline93/1(d), dedisp9/3(we)
  Convert37/1 -> Reinterpret52/1
  Reinterpret52/1 -> dedisp9/2(data_in)
  Counter30/1 -> avg9/1(addr)
  mov_avg9/2(dout_valid) -> Counter30/1, avg9/3(we)
  Convert38/1 -> Reinterpret53/1
  Reinterpret53/1 -> avg9/2(data_in)
  pipeline66/1 -> Register26/3, Register26/1
  Logical40/1 -> pipeline66/1
  Relational14/1 -> Logical40/2
  [rfi_detected] -> Inverter12/1
  Logical41/1 -> Register25/3, Register25/1, enabled_vacc9/1(new_acc)
  acc_cntrl14/1(new_acc) -> Logical41/2
  [en_dedisp] -> Logical41/1
  Register25/1 -> Logical42/1
  [rst_dedisp] -> Register25/2
  Logical42/1 -> enabled_vacc9/3(din_valid)
  pipeline65/1(q) -> Logical42/2
  [detection9] -> Logical3/10
  control/30(acc_len10) -> [acc_len9]
  control/44(theta10) -> [theta9]
  Concat9/1 -> pipeline69/1
  pipeline69/1 -> control/1(frb_detection)
  [rfi_detected] -> control/2(rfi_detected)
  [acc_len10] -> acc_cntrl15/1(acc_len)
  [sd0] -> acc_cntrl15/2(sync)
  [cnt_rst] -> acc_cntrl15/3(rst)
  pipeline70/1(q) -> enabled_vacc10/2(din)
  [m0e10] -> pipeline72/1(d)
  [m0d10] -> pipeline70/1(d)
  enabled_vacc10/1(dout) -> pre_dedisp_conv10/1(din)
  enabled_vacc10/2(dout_valid) -> pre_dedisp_conv10/2(din_valid)
  pre_dedisp_conv10/2(dout_valid) -> pre_dedisp_delay10/2(din_valid)
  pre_dedisp_conv10/1(dout) -> pre_dedisp_delay10/1(In1)
